simulink model "ICAC_AutoSave_20200630_1355"  (R2018b)
(part 2 of 3)

  | T_p_kPa_1_1_u8.Bias = 0;
  | T_p_kPa_1_1_u8.DataTypeOverride = 'Inherit';
  | T_p_kPa_1_1_u8.IsAlias = true;
  | 
  | T_p_kPa_256_1_u16 = Simulink.NumericType;
  | T_p_kPa_256_1_u16.Description = 'kPa (kiloPascals  (kPa))';
  | if (tmpVer > 7.11)
  | 	T_p_kPa_256_1_u16.DataScope = 'Auto';
  | end
  | T_p_kPa_256_1_u16.HeaderFile = 'Rte_Type.h';
  | T_p_kPa_256_1_u16.DataTypeMode = 'Fixed-point: slope and bias scaling';
  | T_p_kPa_256_1_u16.SignednessBool = false;
  | T_p_kPa_256_1_u16.WordLength = 16;
  | T_p_kPa_256_1_u16.FixedExponent = -8;
  | T_p_kPa_256_1_u16.SlopeAdjustmentFactor = 1;
  | T_p_kPa_256_1_u16.Bias = 0;
  | T_p_kPa_256_1_u16.DataTypeOverride = 'Inherit';
  | T_p_kPa_256_1_u16.IsAlias = true;
  | 
  | T_p_kPa_32_1_u16 = Simulink.NumericType;
  | T_p_kPa_32_1_u16.Description = 'kPa (kiloPascals  (kPa))';
  | if (tmpVer > 7.11)
  | 	T_p_kPa_32_1_u16.DataScope = 'Auto';
  | end
  | T_p_kPa_32_1_u16.HeaderFile = 'Rte_Type.h';
  | T_p_kPa_32_1_u16.DataTypeMode = 'Fixed-point: slope and bias scaling';
  | T_p_kPa_32_1_u16.SignednessBool = false;
  | T_p_kPa_32_1_u16.WordLength = 16;
  | T_p_kPa_32_1_u16.FixedExponent = -5;
  | T_p_kPa_32_1_u16.SlopeAdjustmentFactor = 1;
  | T_p_kPa_32_1_u16.Bias = 0;
  | T_p_kPa_32_1_u16.DataTypeOverride = 'Inherit';
  | T_p_kPa_32_1_u16.IsAlias = true;
  | 
  | T_p_kPa_64_1_s16 = Simulink.NumericType;
  | T_p_kPa_64_1_s16.Description = 'kPa (kiloPascals  (kPa))';
  | if (tmpVer > 7.11)
  | 	T_p_kPa_64_1_s16.DataScope = 'Auto';
  | end
  | T_p_kPa_64_1_s16.HeaderFile = 'Rte_Type.h';
  | T_p_kPa_64_1_s16.DataTypeMode = 'Fixed-point: slope and bias scaling';
  | T_p_kPa_64_1_s16.SignednessBool = true;
  | T_p_kPa_64_1_s16.WordLength = 16;
  | T_p_kPa_64_1_s16.FixedExponent = -6;
  | T_p_kPa_64_1_s16.SlopeAdjustmentFactor = 1;
  | T_p_kPa_64_1_s16.Bias = 0;
  | T_p_kPa_64_1_s16.DataTypeOverride = 'Inherit';
  | T_p_kPa_64_1_s16.IsAlias = true;
  | 
  | T_p_kPa_Float32 = Simulink.NumericType;
  | T_p_kPa_Float32.Description = 'kPa (kiloPascals  (kPa))';
  | if (tmpVer > 7.11)
  | 	T_p_kPa_Float32.DataScope = 'Auto';
  | end
  | T_p_kPa_Float32.HeaderFile = 'Rte_Type.h';
  | T_p_kPa_Float32.DataTypeMode = 'Single';
  | T_p_kPa_Float32.SignednessBool = true;
  | T_p_kPa_Float32.WordLength = 32;
  | T_p_kPa_Float32.FixedExponent = 0;
  | T_p_kPa_Float32.SlopeAdjustmentFactor = 1;
  | T_p_kPa_Float32.Bias = 0;
  | T_p_kPa_Float32.DataTypeOverride = 'Inherit';
  | T_p_kPa_Float32.IsAlias = true;
  | 
  | T_phi_deg_100_1_s16 = Simulink.NumericType;
  | T_phi_deg_100_1_s16.Description = 'deg (degrees (deg))';
  | if (tmpVer > 7.11)
  | 	T_phi_deg_100_1_s16.DataScope = 'Auto';
  | end
  | T_phi_deg_100_1_s16.HeaderFile = 'Rte_Type.h';
  | T_phi_deg_100_1_s16.DataTypeMode = ['Fixed-point: slope and bias scalin' ...
  |                                     'g'];
  | T_phi_deg_100_1_s16.SignednessBool = true;
  | T_phi_deg_100_1_s16.WordLength = 16;
  | T_phi_deg_100_1_s16.FixedExponent = -7;
  | T_phi_deg_100_1_s16.SlopeAdjustmentFactor = 1.28;
  | T_phi_deg_100_1_s16.Bias = 0;
  | T_phi_deg_100_1_s16.DataTypeOverride = 'Inherit';
  | T_phi_deg_100_1_s16.IsAlias = true;
  | 
  | T_phi_deg_1024_1_s16 = Simulink.NumericType;
  | T_phi_deg_1024_1_s16.Description = 'deg (degrees (deg))';
  | if (tmpVer > 7.11)
  | 	T_phi_deg_1024_1_s16.DataScope = 'Auto';
  | end
  | T_phi_deg_1024_1_s16.HeaderFile = 'Rte_Type.h';
  | T_phi_deg_1024_1_s16.DataTypeMode = ...
  |   'Fixed-point: slope and bias scaling';
  | T_phi_deg_1024_1_s16.SignednessBool = true;
  | T_phi_deg_1024_1_s16.WordLength = 16;
  | T_phi_deg_1024_1_s16.FixedExponent = -10;
  | T_phi_deg_1024_1_s16.SlopeAdjustmentFactor = 1;
  | T_phi_deg_1024_1_s16.Bias = 0;
  | T_phi_deg_1024_1_s16.DataTypeOverride = 'Inherit';
  | T_phi_deg_1024_1_s16.IsAlias = true;
  | 
  | T_phi_deg_128_1_s16 = Simulink.NumericType;
  | T_phi_deg_128_1_s16.Description = 'deg (degrees (deg))';
  | if (tmpVer > 7.11)
  | 	T_phi_deg_128_1_s16.DataScope = 'Auto';
  | end
  | T_phi_deg_128_1_s16.HeaderFile = 'Rte_Type.h';
  | T_phi_deg_128_1_s16.DataTypeMode = ['Fixed-point: slope and bias scalin' ...
  |                                     'g'];
  | T_phi_deg_128_1_s16.SignednessBool = true;
  | T_phi_deg_128_1_s16.WordLength = 16;
  | T_phi_deg_128_1_s16.FixedExponent = -7;
  | T_phi_deg_128_1_s16.SlopeAdjustmentFactor = 1;
  | T_phi_deg_128_1_s16.Bias = 0;
  | T_phi_deg_128_1_s16.DataTypeOverride = 'Inherit';
  | T_phi_deg_128_1_s16.IsAlias = true;
  | 
  | T_phi_deg_1_1_u8 = Simulink.NumericType;
  | T_phi_deg_1_1_u8.Description = 'deg (degrees (deg))';
  | if (tmpVer > 7.11)
  | 	T_phi_deg_1_1_u8.DataScope = 'Auto';
  | end
  | T_phi_deg_1_1_u8.HeaderFile = 'Rte_Type.h';
  | T_phi_deg_1_1_u8.DataTypeMode = 'Fixed-point: slope and bias scaling';
  | T_phi_deg_1_1_u8.SignednessBool = false;
  | T_phi_deg_1_1_u8.WordLength = 8;
  | T_phi_deg_1_1_u8.FixedExponent = 0;
  | T_phi_deg_1_1_u8.SlopeAdjustmentFactor = 1;
  | T_phi_deg_1_1_u8.Bias = 0;
  | T_phi_deg_1_1_u8.DataTypeOverride = 'Inherit';
  | T_phi_deg_1_1_u8.IsAlias = true;
  | 
  | T_phi_deg_256_1_s16 = Simulink.NumericType;
  | T_phi_deg_256_1_s16.Description = 'deg (degrees (deg))';
  | if (tmpVer > 7.11)
  | 	T_phi_deg_256_1_s16.DataScope = 'Auto';
  | end
  | T_phi_deg_256_1_s16.HeaderFile = 'Rte_Type.h';
  | T_phi_deg_256_1_s16.DataTypeMode = ['Fixed-point: slope and bias scalin' ...
  |                                     'g'];
  | T_phi_deg_256_1_s16.SignednessBool = true;
  | T_phi_deg_256_1_s16.WordLength = 16;
  | T_phi_deg_256_1_s16.FixedExponent = -8;
  | T_phi_deg_256_1_s16.SlopeAdjustmentFactor = 1;
  | T_phi_deg_256_1_s16.Bias = 0;
  | T_phi_deg_256_1_s16.DataTypeOverride = 'Inherit';
  | T_phi_deg_256_1_s16.IsAlias = true;
  | 
  | T_phi_deg_2_1_s8 = Simulink.NumericType;
  | T_phi_deg_2_1_s8.Description = 'deg (degrees (deg))';
  | if (tmpVer > 7.11)
  | 	T_phi_deg_2_1_s8.DataScope = 'Auto';
  | end
  | T_phi_deg_2_1_s8.HeaderFile = 'Rte_Type.h';
  | T_phi_deg_2_1_s8.DataTypeMode = 'Fixed-point: slope and bias scaling';
  | T_phi_deg_2_1_s8.SignednessBool = true;
  | T_phi_deg_2_1_s8.WordLength = 8;
  | T_phi_deg_2_1_s8.FixedExponent = -1;
  | T_phi_deg_2_1_s8.SlopeAdjustmentFactor = 1;
  | T_phi_deg_2_1_s8.Bias = 0;
  | T_phi_deg_2_1_s8.DataTypeOverride = 'Inherit';
  | T_phi_deg_2_1_s8.IsAlias = true;
  | 
  | T_phi_deg_32_1_s16 = Simulink.NumericType;
  | T_phi_deg_32_1_s16.Description = 'deg (degrees (deg))';
  | if (tmpVer > 7.11)
  | 	T_phi_deg_32_1_s16.DataScope = 'Auto';
  | end
  | T_phi_deg_32_1_s16.HeaderFile = 'Rte_Type.h';
  | T_phi_deg_32_1_s16.DataTypeMode = 'Fixed-point: slope and bias scaling';
  | T_phi_deg_32_1_s16.SignednessBool = true;
  | T_phi_deg_32_1_s16.WordLength = 16;
  | T_phi_deg_32_1_s16.FixedExponent = -5;
  | T_phi_deg_32_1_s16.SlopeAdjustmentFactor = 1;
  | T_phi_deg_32_1_s16.Bias = 0;
  | T_phi_deg_32_1_s16.DataTypeOverride = 'Inherit';
  | T_phi_deg_32_1_s16.IsAlias = true;
  | 
  | T_phi_deg_512_6_s32 = Simulink.NumericType;
  | T_phi_deg_512_6_s32.Description = 'deg (degrees (deg))';
  | if (tmpVer > 7.11)
  | 	T_phi_deg_512_6_s32.DataScope = 'Auto';
  | end
  | T_phi_deg_512_6_s32.HeaderFile = 'Rte_Type.h';
  | T_phi_deg_512_6_s32.DataTypeMode = ['Fixed-point: slope and bias scalin' ...
  |                                     'g'];
  | T_phi_deg_512_6_s32.SignednessBool = true;
  | T_phi_deg_512_6_s32.WordLength = 32;
  | T_phi_deg_512_6_s32.FixedExponent = -7;
  | T_phi_deg_512_6_s32.SlopeAdjustmentFactor = 1.5;
  | T_phi_deg_512_6_s32.Bias = 0;
  | T_phi_deg_512_6_s32.DataTypeOverride = 'Inherit';
  | T_phi_deg_512_6_s32.IsAlias = true;
  | 
  | T_phi_deg_Float32 = Simulink.NumericType;
  | T_phi_deg_Float32.Description = 'deg (degrees (deg))';
  | if (tmpVer > 7.11)
  | 	T_phi_deg_Float32.DataScope = 'Auto';
  | end
  | T_phi_deg_Float32.HeaderFile = 'Rte_Type.h';
  | T_phi_deg_Float32.DataTypeMode = 'Single';
  | T_phi_deg_Float32.SignednessBool = true;
  | T_phi_deg_Float32.WordLength = 32;
  | T_phi_deg_Float32.FixedExponent = 0;
  | T_phi_deg_Float32.SlopeAdjustmentFactor = 1;
  | T_phi_deg_Float32.Bias = 0;
  | T_phi_deg_Float32.DataTypeOverride = 'Inherit';
  | T_phi_deg_Float32.IsAlias = true;
  | 
  | T_phi_rad_2048_1_s16 = Simulink.NumericType;
  | T_phi_rad_2048_1_s16.Description = 'rad (radians  (rad))';
  | if (tmpVer > 7.11)
  | 	T_phi_rad_2048_1_s16.DataScope = 'Auto';
  | end
  | T_phi_rad_2048_1_s16.HeaderFile = 'Rte_Type.h';
  | T_phi_rad_2048_1_s16.DataTypeMode = ...
  |   'Fixed-point: slope and bias scaling';
  | T_phi_rad_2048_1_s16.SignednessBool = true;
  | T_phi_rad_2048_1_s16.WordLength = 16;
  | T_phi_rad_2048_1_s16.FixedExponent = -11;
  | T_phi_rad_2048_1_s16.SlopeAdjustmentFactor = 1;
  | T_phi_rad_2048_1_s16.Bias = 0;
  | T_phi_rad_2048_1_s16.DataTypeOverride = 'Inherit';
  | T_phi_rad_2048_1_s16.IsAlias = true;
  | 
  | T_phi_rad_Float32 = Simulink.NumericType;
  | T_phi_rad_Float32.Description = 'rad (radians  (rad))';
  | if (tmpVer > 7.11)
  | 	T_phi_rad_Float32.DataScope = 'Auto';
  | end
  | T_phi_rad_Float32.HeaderFile = 'Rte_Type.h';
  | T_phi_rad_Float32.DataTypeMode = 'Single';
  | T_phi_rad_Float32.SignednessBool = true;
  | T_phi_rad_Float32.WordLength = 32;
  | T_phi_rad_Float32.FixedExponent = 0;
  | T_phi_rad_Float32.SlopeAdjustmentFactor = 1;
  | T_phi_rad_Float32.Bias = 0;
  | T_phi_rad_Float32.DataTypeOverride = 'Inherit';
  | T_phi_rad_Float32.IsAlias = true;
  | 
  | T_r_NA_1024_1_s16 = Simulink.NumericType;
  | T_r_NA_1024_1_s16.Description = 'NA (none)';
  | if (tmpVer > 7.11)
  | 	T_r_NA_1024_1_s16.DataScope = 'Auto';
  | end
  | T_r_NA_1024_1_s16.HeaderFile = 'Rte_Type.h';
  | T_r_NA_1024_1_s16.DataTypeMode = 'Fixed-point: slope and bias scaling';
  | T_r_NA_1024_1_s16.SignednessBool = true;
  | T_r_NA_1024_1_s16.WordLength = 16;
  | T_r_NA_1024_1_s16.FixedExponent = -10;
  | T_r_NA_1024_1_s16.SlopeAdjustmentFactor = 1;
  | T_r_NA_1024_1_s16.Bias = 0;
  | T_r_NA_1024_1_s16.DataTypeOverride = 'Inherit';
  | T_r_NA_1024_1_s16.IsAlias = true;
  | 
  | T_r_NA_1024_1_u16 = Simulink.NumericType;
  | T_r_NA_1024_1_u16.Description = 'NA (none)';
  | if (tmpVer > 7.11)
  | 	T_r_NA_1024_1_u16.DataScope = 'Auto';
  | end
  | T_r_NA_1024_1_u16.HeaderFile = 'Rte_Type.h';
  | T_r_NA_1024_1_u16.DataTypeMode = 'Fixed-point: slope and bias scaling';
  | T_r_NA_1024_1_u16.SignednessBool = false;
  | T_r_NA_1024_1_u16.WordLength = 16;
  | T_r_NA_1024_1_u16.FixedExponent = -10;
  | T_r_NA_1024_1_u16.SlopeAdjustmentFactor = 1;
  | T_r_NA_1024_1_u16.Bias = 0;
  | T_r_NA_1024_1_u16.DataTypeOverride = 'Inherit';
  | T_r_NA_1024_1_u16.IsAlias = true;
  | 
  | T_r_NA_16384_1_s16 = Simulink.NumericType;
  | T_r_NA_16384_1_s16.Description = 'NA (none)';
  | if (tmpVer > 7.11)
  | 	T_r_NA_16384_1_s16.DataScope = 'Auto';
  | end
  | T_r_NA_16384_1_s16.HeaderFile = 'Rte_Type.h';
  | T_r_NA_16384_1_s16.DataTypeMode = 'Fixed-point: slope and bias scaling';
  | T_r_NA_16384_1_s16.SignednessBool = true;
  | T_r_NA_16384_1_s16.WordLength = 16;
  | T_r_NA_16384_1_s16.FixedExponent = -14;
  | T_r_NA_16384_1_s16.SlopeAdjustmentFactor = 1;
  | T_r_NA_16384_1_s16.Bias = 0;
  | T_r_NA_16384_1_s16.DataTypeOverride = 'Inherit';
  | T_r_NA_16384_1_s16.IsAlias = true;
  | 
  | T_r_NA_16_1_s16 = Simulink.NumericType;
  | T_r_NA_16_1_s16.Description = 'NA (none)';
  | if (tmpVer > 7.11)
  | 	T_r_NA_16_1_s16.DataScope = 'Auto';
  | end
  | T_r_NA_16_1_s16.HeaderFile = 'Rte_Type.h';
  | T_r_NA_16_1_s16.DataTypeMode = 'Fixed-point: slope and bias scaling';
  | T_r_NA_16_1_s16.SignednessBool = true;
  | T_r_NA_16_1_s16.WordLength = 16;
  | T_r_NA_16_1_s16.FixedExponent = -4;
  | T_r_NA_16_1_s16.SlopeAdjustmentFactor = 1;
  | T_r_NA_16_1_s16.Bias = 0;
  | T_r_NA_16_1_s16.DataTypeOverride = 'Inherit';
  | T_r_NA_16_1_s16.IsAlias = true;
  | 
  | T_r_NA_256_1_s8 = Simulink.NumericType;
  | T_r_NA_256_1_s8.Description = 'NA (none)';
  | if (tmpVer > 7.11)
  | 	T_r_NA_256_1_s8.DataScope = 'Auto';
  | end
  | T_r_NA_256_1_s8.HeaderFile = 'Rte_Type.h';
  | T_r_NA_256_1_s8.DataTypeMode = 'Fixed-point: slope and bias scaling';
  | T_r_NA_256_1_s8.SignednessBool = true;
  | T_r_NA_256_1_s8.WordLength = 8;
  | T_r_NA_256_1_s8.FixedExponent = -8;
  | T_r_NA_256_1_s8.SlopeAdjustmentFactor = 1;
  | T_r_NA_256_1_s8.Bias = 0;
  | T_r_NA_256_1_s8.DataTypeOverride = 'Inherit';
  | T_r_NA_256_1_s8.IsAlias = true;
  | 
  | T_r_NA_256_1_u16 = Simulink.NumericType;
  | T_r_NA_256_1_u16.Description = 'NA (none)';
  | if (tmpVer > 7.11)
  | 	T_r_NA_256_1_u16.DataScope = 'Auto';
  | end
  | T_r_NA_256_1_u16.HeaderFile = 'Rte_Type.h';
  | T_r_NA_256_1_u16.DataTypeMode = 'Fixed-point: slope and bias scaling';
  | T_r_NA_256_1_u16.SignednessBool = false;
  | T_r_NA_256_1_u16.WordLength = 16;
  | T_r_NA_256_1_u16.FixedExponent = -8;
  | T_r_NA_256_1_u16.SlopeAdjustmentFactor = 1;
  | T_r_NA_256_1_u16.Bias = 0;
  | T_r_NA_256_1_u16.DataTypeOverride = 'Inherit';
  | T_r_NA_256_1_u16.IsAlias = true;
  | 
  | T_r_NA_32768_1_u16 = Simulink.NumericType;
  | T_r_NA_32768_1_u16.Description = 'NA (none)';
  | if (tmpVer > 7.11)
  | 	T_r_NA_32768_1_u16.DataScope = 'Auto';
  | end
  | T_r_NA_32768_1_u16.HeaderFile = 'Rte_Type.h';
  | T_r_NA_32768_1_u16.DataTypeMode = 'Fixed-point: slope and bias scaling';
  | T_r_NA_32768_1_u16.SignednessBool = false;
  | T_r_NA_32768_1_u16.WordLength = 16;
  | T_r_NA_32768_1_u16.FixedExponent = -15;
  | T_r_NA_32768_1_u16.SlopeAdjustmentFactor = 1;
  | T_r_NA_32768_1_u16.Bias = 0;
  | T_r_NA_32768_1_u16.DataTypeOverride = 'Inherit';
  | T_r_NA_32768_1_u16.IsAlias = true;
  | 
  | T_r_NA_32_1_u16 = Simulink.NumericType;
  | T_r_NA_32_1_u16.Description = 'NA (none)';
  | if (tmpVer > 7.11)
  | 	T_r_NA_32_1_u16.DataScope = 'Auto';
  | end
  | T_r_NA_32_1_u16.HeaderFile = 'Rte_Type.h';
  | T_r_NA_32_1_u16.DataTypeMode = 'Fixed-point: slope and bias scaling';
  | T_r_NA_32_1_u16.SignednessBool = false;
  | T_r_NA_32_1_u16.WordLength = 16;
  | T_r_NA_32_1_u16.FixedExponent = -5;
  | T_r_NA_32_1_u16.SlopeAdjustmentFactor = 1;
  | T_r_NA_32_1_u16.Bias = 0;
  | T_r_NA_32_1_u16.DataTypeOverride = 'Inherit';
  | T_r_NA_32_1_u16.IsAlias = true;
  | 
  | T_r_NA_4096_1_s16 = Simulink.NumericType;
  | T_r_NA_4096_1_s16.Description = 'NA (none)';
  | if (tmpVer > 7.11)
  | 	T_r_NA_4096_1_s16.DataScope = 'Auto';
  | end
  | T_r_NA_4096_1_s16.HeaderFile = 'Rte_Type.h';
  | T_r_NA_4096_1_s16.DataTypeMode = 'Fixed-point: slope and bias scaling';
  | T_r_NA_4096_1_s16.SignednessBool = true;
  | T_r_NA_4096_1_s16.WordLength = 16;
  | T_r_NA_4096_1_s16.FixedExponent = -12;
  | T_r_NA_4096_1_s16.SlopeAdjustmentFactor = 1;
  | T_r_NA_4096_1_s16.Bias = 0;
  | T_r_NA_4096_1_s16.DataTypeOverride = 'Inherit';
  | T_r_NA_4096_1_s16.IsAlias = true;
  | 
  | T_r_NA_65535_2_u16 = Simulink.NumericType;
  | T_r_NA_65535_2_u16.Description = 'NA (none)';
  | if (tmpVer > 7.11)
  | 	T_r_NA_65535_2_u16.DataScope = 'Auto';
  | end
  | T_r_NA_65535_2_u16.HeaderFile = 'Rte_Type.h';
  | T_r_NA_65535_2_u16.DataTypeMode = 'Fixed-point: slope and bias scaling';
  | T_r_NA_65535_2_u16.SignednessBool = false;
  | T_r_NA_65535_2_u16.WordLength = 16;
  | T_r_NA_65535_2_u16.FixedExponent = -15;
  | T_r_NA_65535_2_u16.SlopeAdjustmentFactor = 1.0000152590218967;
  | T_r_NA_65535_2_u16.Bias = 0;
  | T_r_NA_65535_2_u16.DataTypeOverride = 'Inherit';
  | T_r_NA_65535_2_u16.IsAlias = true;
  | 
  | T_r_NA_8192_1_u16 = Simulink.NumericType;
  | T_r_NA_8192_1_u16.Description = 'NA (none)';
  | if (tmpVer > 7.11)
  | 	T_r_NA_8192_1_u16.DataScope = 'Auto';
  | end
  | T_r_NA_8192_1_u16.HeaderFile = 'Rte_Type.h';
  | T_r_NA_8192_1_u16.DataTypeMode = 'Fixed-point: slope and bias scaling';
  | T_r_NA_8192_1_u16.SignednessBool = false;
  | T_r_NA_8192_1_u16.WordLength = 16;
  | T_r_NA_8192_1_u16.FixedExponent = -13;
  | T_r_NA_8192_1_u16.SlopeAdjustmentFactor = 1;
  | T_r_NA_8192_1_u16.Bias = 0;
  | T_r_NA_8192_1_u16.DataTypeOverride = 'Inherit';
  | T_r_NA_8192_1_u16.IsAlias = true;
  | 
  | T_r_NA_Float32 = Simulink.NumericType;
  | T_r_NA_Float32.Description = 'NA (none)';
  | if (tmpVer > 7.11)
  | 	T_r_NA_Float32.DataScope = 'Auto';
  | end
  | T_r_NA_Float32.HeaderFile = 'Rte_Type.h';
  | T_r_NA_Float32.DataTypeMode = 'Single';
  | T_r_NA_Float32.SignednessBool = true;
  | T_r_NA_Float32.WordLength = 32;
  | T_r_NA_Float32.FixedExponent = 0;
  | T_r_NA_Float32.SlopeAdjustmentFactor = 1;
  | T_r_NA_Float32.Bias = 0;
  | T_r_NA_Float32.DataTypeOverride = 'Inherit';
  | T_r_NA_Float32.IsAlias = true;
  | 
  | T_rho_gpl_8192_1_s16 = Simulink.NumericType;
  | T_rho_gpl_8192_1_s16.Description = 'gpl (grams / liter  (g/l))';
  | if (tmpVer > 7.11)
  | 	T_rho_gpl_8192_1_s16.DataScope = 'Auto';
  | end
  | T_rho_gpl_8192_1_s16.HeaderFile = 'Rte_Type.h';
  | T_rho_gpl_8192_1_s16.DataTypeMode = ...
  |   'Fixed-point: slope and bias scaling';
  | T_rho_gpl_8192_1_s16.SignednessBool = true;
  | T_rho_gpl_8192_1_s16.WordLength = 16;
  | T_rho_gpl_8192_1_s16.FixedExponent = -13;
  | T_rho_gpl_8192_1_s16.SlopeAdjustmentFactor = 1;
  | T_rho_gpl_8192_1_s16.Bias = 0;
  | T_rho_gpl_8192_1_s16.DataTypeOverride = 'Inherit';
  | T_rho_gpl_8192_1_s16.IsAlias = true;
  | 
  | T_rho_gpl_Float32 = Simulink.NumericType;
  | T_rho_gpl_Float32.Description = 'gpl (grams / liter  (g/l))';
  | if (tmpVer > 7.11)
  | 	T_rho_gpl_Float32.DataScope = 'Auto';
  | end
  | T_rho_gpl_Float32.HeaderFile = 'Rte_Type.h';
  | T_rho_gpl_Float32.DataTypeMode = 'Single';
  | T_rho_gpl_Float32.SignednessBool = true;
  | T_rho_gpl_Float32.WordLength = 32;
  | T_rho_gpl_Float32.FixedExponent = 0;
  | T_rho_gpl_Float32.SlopeAdjustmentFactor = 1;
  | T_rho_gpl_Float32.Bias = 0;
  | T_rho_gpl_Float32.DataTypeOverride = 'Inherit';
  | T_rho_gpl_Float32.IsAlias = true;
  | 
  | T_rho_kgpm3_16_1_s16 = Simulink.NumericType;
  | T_rho_kgpm3_16_1_s16.Description = ['kgpm3 (kilograms / cubic meter  (k' ...
  |                                     'g/m3))'];
  | if (tmpVer > 7.11)
  | 	T_rho_kgpm3_16_1_s16.DataScope = 'Auto';
  | end
  | T_rho_kgpm3_16_1_s16.HeaderFile = 'Rte_Type.h';
  | T_rho_kgpm3_16_1_s16.DataTypeMode = ...
  |   'Fixed-point: slope and bias scaling';
  | T_rho_kgpm3_16_1_s16.SignednessBool = true;
  | T_rho_kgpm3_16_1_s16.WordLength = 16;
  | T_rho_kgpm3_16_1_s16.FixedExponent = -4;
  | T_rho_kgpm3_16_1_s16.SlopeAdjustmentFactor = 1;
  | T_rho_kgpm3_16_1_s16.Bias = 0;
  | T_rho_kgpm3_16_1_s16.DataTypeOverride = 'Inherit';
  | T_rho_kgpm3_16_1_s16.IsAlias = true;
  | 
  | T_rho_kgpm3_Float32 = Simulink.NumericType;
  | T_rho_kgpm3_Float32.Description = ['kgpm3 (kilograms / cubic meter  (kg' ...
  |                                    '/m3))'];
  | if (tmpVer > 7.11)
  | 	T_rho_kgpm3_Float32.DataScope = 'Auto';
  | end
  | T_rho_kgpm3_Float32.HeaderFile = 'Rte_Type.h';
  | T_rho_kgpm3_Float32.DataTypeMode = 'Single';
  | T_rho_kgpm3_Float32.SignednessBool = true;
  | T_rho_kgpm3_Float32.WordLength = 32;
  | T_rho_kgpm3_Float32.FixedExponent = 0;
  | T_rho_kgpm3_Float32.SlopeAdjustmentFactor = 1;
  | T_rho_kgpm3_Float32.Bias = 0;
  | T_rho_kgpm3_Float32.DataTypeOverride = 'Inherit';
  | T_rho_kgpm3_Float32.IsAlias = true;
  | 
  | T_rho_mgpl_1_1_s16 = Simulink.NumericType;
  | T_rho_mgpl_1_1_s16.Description = 'mgpl (milligrams / liter  (mg/l))';
  | if (tmpVer > 7.11)
  | 	T_rho_mgpl_1_1_s16.DataScope = 'Auto';
  | end
  | T_rho_mgpl_1_1_s16.HeaderFile = 'Rte_Type.h';
  | T_rho_mgpl_1_1_s16.DataTypeMode = 'Fixed-point: slope and bias scaling';
  | T_rho_mgpl_1_1_s16.SignednessBool = true;
  | T_rho_mgpl_1_1_s16.WordLength = 16;
  | T_rho_mgpl_1_1_s16.FixedExponent = 0;
  | T_rho_mgpl_1_1_s16.SlopeAdjustmentFactor = 1;
  | T_rho_mgpl_1_1_s16.Bias = 0;
  | T_rho_mgpl_1_1_s16.DataTypeOverride = 'Inherit';
  | T_rho_mgpl_1_1_s16.IsAlias = true;
  | 
  | T_rho_mgpl_64_1_s16 = Simulink.NumericType;
  | T_rho_mgpl_64_1_s16.Description = 'mgpl (milligrams / liter  (mg/l))';
  | if (tmpVer > 7.11)
  | 	T_rho_mgpl_64_1_s16.DataScope = 'Auto';
  | end
  | T_rho_mgpl_64_1_s16.HeaderFile = 'Rte_Type.h';
  | T_rho_mgpl_64_1_s16.DataTypeMode = ['Fixed-point: slope and bias scalin' ...
  |                                     'g'];
  | T_rho_mgpl_64_1_s16.SignednessBool = true;
  | T_rho_mgpl_64_1_s16.WordLength = 16;
  | T_rho_mgpl_64_1_s16.FixedExponent = -6;
  | T_rho_mgpl_64_1_s16.SlopeAdjustmentFactor = 1;
  | T_rho_mgpl_64_1_s16.Bias = 0;
  | T_rho_mgpl_64_1_s16.DataTypeOverride = 'Inherit';
  | T_rho_mgpl_64_1_s16.IsAlias = true;
  | 
  | T_rho_mgpl_Float32 = Simulink.NumericType;
  | T_rho_mgpl_Float32.Description = 'mgpl (milligrams / liter  (mg/l))';
  | if (tmpVer > 7.11)
  | 	T_rho_mgpl_Float32.DataScope = 'Auto';
  | end
  | T_rho_mgpl_Float32.HeaderFile = 'Rte_Type.h';
  | T_rho_mgpl_Float32.DataTypeMode = 'Single';
  | T_rho_mgpl_Float32.SignednessBool = true;
  | T_rho_mgpl_Float32.WordLength = 32;
  | T_rho_mgpl_Float32.FixedExponent = 0;
  | T_rho_mgpl_Float32.SlopeAdjustmentFactor = 1;
  | T_rho_mgpl_Float32.Bias = 0;
  | T_rho_mgpl_Float32.DataTypeOverride = 'Inherit';
  | T_rho_mgpl_Float32.IsAlias = true;
  | 
  | T_t_hour_1_1_s16 = Simulink.NumericType;
  | T_t_hour_1_1_s16.Description = 'h (hour  (h))';
  | if (tmpVer > 7.11)
  | 	T_t_hour_1_1_s16.DataScope = 'Auto';
  | end
  | T_t_hour_1_1_s16.HeaderFile = 'Rte_Type.h';
  | T_t_hour_1_1_s16.DataTypeMode = 'Fixed-point: slope and bias scaling';
  | T_t_hour_1_1_s16.SignednessBool = true;
  | T_t_hour_1_1_s16.WordLength = 16;
  | T_t_hour_1_1_s16.FixedExponent = 0;
  | T_t_hour_1_1_s16.SlopeAdjustmentFactor = 1;
  | T_t_hour_1_1_s16.Bias = 0;
  | T_t_hour_1_1_s16.DataTypeOverride = 'Inherit';
  | T_t_hour_1_1_s16.IsAlias = true;
  | 
  | T_t_hour_Float32 = Simulink.NumericType;
  | T_t_hour_Float32.Description = 'h (hour  (h))';
  | if (tmpVer > 7.11)
  | 	T_t_hour_Float32.DataScope = 'Auto';
  | end
  | T_t_hour_Float32.HeaderFile = 'Rte_Type.h';
  | T_t_hour_Float32.DataTypeMode = 'Single';
  | T_t_hour_Float32.SignednessBool = true;
  | T_t_hour_Float32.WordLength = 32;
  | T_t_hour_Float32.FixedExponent = 0;
  | T_t_hour_Float32.SlopeAdjustmentFactor = 1;
  | T_t_hour_Float32.Bias = 0;
  | T_t_hour_Float32.DataTypeOverride = 'Inherit';
  | T_t_hour_Float32.IsAlias = true;
  | 
  | T_t_m_1_1_u16 = Simulink.NumericType;
  | T_t_m_1_1_u16.Description = 'm (minutes  (m))';
  | if (tmpVer > 7.11)
  | 	T_t_m_1_1_u16.DataScope = 'Auto';
  | end
  | T_t_m_1_1_u16.HeaderFile = 'Rte_Type.h';
  | T_t_m_1_1_u16.DataTypeMode = 'Fixed-point: slope and bias scaling';
  | T_t_m_1_1_u16.SignednessBool = false;
  | T_t_m_1_1_u16.WordLength = 16;
  | T_t_m_1_1_u16.FixedExponent = 0;
  | T_t_m_1_1_u16.SlopeAdjustmentFactor = 1;
  | T_t_m_1_1_u16.Bias = 0;
  | T_t_m_1_1_u16.DataTypeOverride = 'Inherit';
  | T_t_m_1_1_u16.IsAlias = true;
  | 
  | T_t_m_Float32 = Simulink.NumericType;
  | T_t_m_Float32.Description = 'm (minutes  (m))';
  | if (tmpVer > 7.11)
  | 	T_t_m_Float32.DataScope = 'Auto';
  | end
  | T_t_m_Float32.HeaderFile = 'Rte_Type.h';
  | T_t_m_Float32.DataTypeMode = 'Single';
  | T_t_m_Float32.SignednessBool = true;
  | T_t_m_Float32.WordLength = 32;
  | T_t_m_Float32.FixedExponent = 0;
  | T_t_m_Float32.SlopeAdjustmentFactor = 1;
  | T_t_m_Float32.Bias = 0;
  | T_t_m_Float32.DataTypeOverride = 'Inherit';
  | T_t_m_Float32.IsAlias = true;
  | 
  | T_t_ms_1_1_s16 = Simulink.NumericType;
  | T_t_ms_1_1_s16.Description = 'ms (milliseconds  (ms))';
  | if (tmpVer > 7.11)
  | 	T_t_ms_1_1_s16.DataScope = 'Auto';
  | end
  | T_t_ms_1_1_s16.HeaderFile = 'Rte_Type.h';
  | T_t_ms_1_1_s16.DataTypeMode = 'Fixed-point: slope and bias scaling';
  | T_t_ms_1_1_s16.SignednessBool = true;
  | T_t_ms_1_1_s16.WordLength = 16;
  | T_t_ms_1_1_s16.FixedExponent = 0;
  | T_t_ms_1_1_s16.SlopeAdjustmentFactor = 1;
  | T_t_ms_1_1_s16.Bias = 0;
  | T_t_ms_1_1_s16.DataTypeOverride = 'Inherit';
  | T_t_ms_1_1_s16.IsAlias = true;
  | 
  | T_t_ms_1_1_u16 = Simulink.NumericType;
  | T_t_ms_1_1_u16.Description = 'ms (milliseconds  (ms))';
  | if (tmpVer > 7.11)
  | 	T_t_ms_1_1_u16.DataScope = 'Auto';
  | end
  | T_t_ms_1_1_u16.HeaderFile = 'Rte_Type.h';
  | T_t_ms_1_1_u16.DataTypeMode = 'Fixed-point: slope and bias scaling';
  | T_t_ms_1_1_u16.SignednessBool = false;
  | T_t_ms_1_1_u16.WordLength = 16;
  | T_t_ms_1_1_u16.FixedExponent = 0;
  | T_t_ms_1_1_u16.SlopeAdjustmentFactor = 1;
  | T_t_ms_1_1_u16.Bias = 0;
  | T_t_ms_1_1_u16.DataTypeOverride = 'Inherit';
  | T_t_ms_1_1_u16.IsAlias = true;
  | 
  | T_t_ms_1_1_u32 = Simulink.NumericType;
  | T_t_ms_1_1_u32.Description = 'ms (milliseconds  (ms))';
  | if (tmpVer > 7.11)
  | 	T_t_ms_1_1_u32.DataScope = 'Auto';
  | end
  | T_t_ms_1_1_u32.HeaderFile = 'Rte_Type.h';
  | T_t_ms_1_1_u32.DataTypeMode = 'Fixed-point: slope and bias scaling';
  | T_t_ms_1_1_u32.SignednessBool = false;
  | T_t_ms_1_1_u32.WordLength = 32;
  | T_t_ms_1_1_u32.FixedExponent = 0;
  | T_t_ms_1_1_u32.SlopeAdjustmentFactor = 1;
  | T_t_ms_1_1_u32.Bias = 0;
  | T_t_ms_1_1_u32.DataTypeOverride = 'Inherit';
  | T_t_ms_1_1_u32.IsAlias = true;
  | 
  | T_t_ms_4096_1_s16 = Simulink.NumericType;
  | T_t_ms_4096_1_s16.Description = 'ms (milliseconds  (ms))';
  | if (tmpVer > 7.11)
  | 	T_t_ms_4096_1_s16.DataScope = 'Auto';
  | end
  | T_t_ms_4096_1_s16.HeaderFile = 'Rte_Type.h';
  | T_t_ms_4096_1_s16.DataTypeMode = 'Fixed-point: slope and bias scaling';
  | T_t_ms_4096_1_s16.SignednessBool = true;
  | T_t_ms_4096_1_s16.WordLength = 16;
  | T_t_ms_4096_1_s16.FixedExponent = -12;
  | T_t_ms_4096_1_s16.SlopeAdjustmentFactor = 1;
  | T_t_ms_4096_1_s16.Bias = 0;
  | T_t_ms_4096_1_s16.DataTypeOverride = 'Inherit';
  | T_t_ms_4096_1_s16.IsAlias = true;
  | 
  | T_t_ms_64_1_s16 = Simulink.NumericType;
  | T_t_ms_64_1_s16.Description = 'ms (milliseconds  (ms))';
  | if (tmpVer > 7.11)
  | 	T_t_ms_64_1_s16.DataScope = 'Auto';
  | end
  | T_t_ms_64_1_s16.HeaderFile = 'Rte_Type.h';
  | T_t_ms_64_1_s16.DataTypeMode = 'Fixed-point: slope and bias scaling';
  | T_t_ms_64_1_s16.SignednessBool = true;
  | T_t_ms_64_1_s16.WordLength = 16;
  | T_t_ms_64_1_s16.FixedExponent = -6;
  | T_t_ms_64_1_s16.SlopeAdjustmentFactor = 1;
  | T_t_ms_64_1_s16.Bias = 0;
  | T_t_ms_64_1_s16.DataTypeOverride = 'Inherit';
  | T_t_ms_64_1_s16.IsAlias = true;
  | 
  | T_t_ms_Float32 = Simulink.NumericType;
  | T_t_ms_Float32.Description = 'ms (milliseconds  (ms))';
  | if (tmpVer > 7.11)
  | 	T_t_ms_Float32.DataScope = 'Auto';
  | end
  | T_t_ms_Float32.HeaderFile = 'Rte_Type.h';
  | T_t_ms_Float32.DataTypeMode = 'Single';
  | T_t_ms_Float32.SignednessBool = true;
  | T_t_ms_Float32.WordLength = 32;
  | T_t_ms_Float32.FixedExponent = 0;
  | T_t_ms_Float32.SlopeAdjustmentFactor = 1;
  | T_t_ms_Float32.Bias = 0;
  | T_t_ms_Float32.DataTypeOverride = 'Inherit';
  | T_t_ms_Float32.IsAlias = true;
  | 
  | T_t_s_1000_1_s16 = Simulink.NumericType;
  | T_t_s_1000_1_s16.Description = 's (seconds  (s))';
  | if (tmpVer > 7.11)
  | 	T_t_s_1000_1_s16.DataScope = 'Auto';
  | end
  | T_t_s_1000_1_s16.HeaderFile = 'Rte_Type.h';
  | T_t_s_1000_1_s16.DataTypeMode = 'Fixed-point: slope and bias scaling';
  | T_t_s_1000_1_s16.SignednessBool = true;
  | T_t_s_1000_1_s16.WordLength = 16;
  | T_t_s_1000_1_s16.FixedExponent = -10;
  | T_t_s_1000_1_s16.SlopeAdjustmentFactor = 1.024;
  | T_t_s_1000_1_s16.Bias = 0;
  | T_t_s_1000_1_s16.DataTypeOverride = 'Inherit';
  | T_t_s_1000_1_s16.IsAlias = true;
  | 
  | T_t_s_100_1_s16 = Simulink.NumericType;
  | T_t_s_100_1_s16.Description = 's (seconds  (s))';
  | if (tmpVer > 7.11)
  | 	T_t_s_100_1_s16.DataScope = 'Auto';
  | end
  | T_t_s_100_1_s16.HeaderFile = 'Rte_Type.h';
  | T_t_s_100_1_s16.DataTypeMode = 'Fixed-point: slope and bias scaling';
  | T_t_s_100_1_s16.SignednessBool = true;
  | T_t_s_100_1_s16.WordLength = 16;
  | T_t_s_100_1_s16.FixedExponent = -7;
  | T_t_s_100_1_s16.SlopeAdjustmentFactor = 1.28;
  | T_t_s_100_1_s16.Bias = 0;
  | T_t_s_100_1_s16.DataTypeOverride = 'Inherit';
  | T_t_s_100_1_s16.IsAlias = true;
  | 
  | T_t_s_10_1_s16 = Simulink.NumericType;
  | T_t_s_10_1_s16.Description = 's (seconds  (s))';
  | if (tmpVer > 7.11)
  | 	T_t_s_10_1_s16.DataScope = 'Auto';
  | end
  | T_t_s_10_1_s16.HeaderFile = 'Rte_Type.h';
  | T_t_s_10_1_s16.DataTypeMode = 'Fixed-point: slope and bias scaling';
  | T_t_s_10_1_s16.SignednessBool = true;
  | T_t_s_10_1_s16.WordLength = 16;
  | T_t_s_10_1_s16.FixedExponent = -4;
  | T_t_s_10_1_s16.SlopeAdjustmentFactor = 1.6;
  | T_t_s_10_1_s16.Bias = 0;
  | T_t_s_10_1_s16.DataTypeOverride = 'Inherit';
  | T_t_s_10_1_s16.IsAlias = true;
  | 
  | T_t_s_10_1_u16 = Simulink.NumericType;
  | T_t_s_10_1_u16.Description = 's (seconds  (s))';
  | if (tmpVer > 7.11)
  | 	T_t_s_10_1_u16.DataScope = 'Auto';
  | end
  | T_t_s_10_1_u16.HeaderFile = 'Rte_Type.h';
  | T_t_s_10_1_u16.DataTypeMode = 'Fixed-point: slope and bias scaling';
  | T_t_s_10_1_u16.SignednessBool = false;
  | T_t_s_10_1_u16.WordLength = 16;
  | T_t_s_10_1_u16.FixedExponent = -4;
  | T_t_s_10_1_u16.SlopeAdjustmentFactor = 1.6;
  | T_t_s_10_1_u16.Bias = 0;
  | T_t_s_10_1_u16.DataTypeOverride = 'Inherit';
  | T_t_s_10_1_u16.IsAlias = true;
  | 
  | T_t_s_1_1_s16 = Simulink.NumericType;
  | T_t_s_1_1_s16.Description = 's (seconds  (s))';
  | if (tmpVer > 7.11)
  | 	T_t_s_1_1_s16.DataScope = 'Auto';
  | end
  | T_t_s_1_1_s16.HeaderFile = 'Rte_Type.h';
  | T_t_s_1_1_s16.DataTypeMode = 'Fixed-point: slope and bias scaling';
  | T_t_s_1_1_s16.SignednessBool = true;
  | T_t_s_1_1_s16.WordLength = 16;
  | T_t_s_1_1_s16.FixedExponent = 0;
  | T_t_s_1_1_s16.SlopeAdjustmentFactor = 1;
  | T_t_s_1_1_s16.Bias = 0;
  | T_t_s_1_1_s16.DataTypeOverride = 'Inherit';
  | T_t_s_1_1_s16.IsAlias = true;
  | 
  | T_t_s_1_1_u16 = Simulink.NumericType;
  | T_t_s_1_1_u16.Description = 's (seconds  (s))';
  | if (tmpVer > 7.11)
  | 	T_t_s_1_1_u16.DataScope = 'Auto';
  | end
  | T_t_s_1_1_u16.HeaderFile = 'Rte_Type.h';
  | T_t_s_1_1_u16.DataTypeMode = 'Fixed-point: slope and bias scaling';
  | T_t_s_1_1_u16.SignednessBool = false;
  | T_t_s_1_1_u16.WordLength = 16;
  | T_t_s_1_1_u16.FixedExponent = 0;
  | T_t_s_1_1_u16.SlopeAdjustmentFactor = 1;
  | T_t_s_1_1_u16.Bias = 0;
  | T_t_s_1_1_u16.DataTypeOverride = 'Inherit';
  | T_t_s_1_1_u16.IsAlias = true;
  | 
  | T_t_s_1_1_u32 = Simulink.NumericType;
  | T_t_s_1_1_u32.Description = 's (seconds  (s))';
  | if (tmpVer > 7.11)
  | 	T_t_s_1_1_u32.DataScope = 'Auto';
  | end
  | T_t_s_1_1_u32.HeaderFile = 'Rte_Type.h';
  | T_t_s_1_1_u32.DataTypeMode = 'Fixed-point: slope and bias scaling';
  | T_t_s_1_1_u32.SignednessBool = false;
  | T_t_s_1_1_u32.WordLength = 32;
  | T_t_s_1_1_u32.FixedExponent = 0;
  | T_t_s_1_1_u32.SlopeAdjustmentFactor = 1;
  | T_t_s_1_1_u32.Bias = 0;
  | T_t_s_1_1_u32.DataTypeOverride = 'Inherit';
  | T_t_s_1_1_u32.IsAlias = true;
  | 
  | T_t_s_Float32 = Simulink.NumericType;
  | T_t_s_Float32.Description = 's (seconds  (s))';
  | if (tmpVer > 7.11)
  | 	T_t_s_Float32.DataScope = 'Auto';
  | end
  | T_t_s_Float32.HeaderFile = 'Rte_Type.h';
  | T_t_s_Float32.DataTypeMode = 'Single';
  | T_t_s_Float32.SignednessBool = true;
  | T_t_s_Float32.WordLength = 32;
  | T_t_s_Float32.FixedExponent = 0;
  | T_t_s_Float32.SlopeAdjustmentFactor = 1;
  | T_t_s_Float32.Bias = 0;
  | T_t_s_Float32.DataTypeOverride = 'Inherit';
  | T_t_s_Float32.IsAlias = true;
  | 
  | T_t_us_10_1_u32 = Simulink.NumericType;
  | T_t_us_10_1_u32.Description = 'us (microseconds  (us))';
  | if (tmpVer > 7.11)
  | 	T_t_us_10_1_u32.DataScope = 'Auto';
  | end
  | T_t_us_10_1_u32.HeaderFile = 'Rte_Type.h';
  | T_t_us_10_1_u32.DataTypeMode = 'Fixed-point: slope and bias scaling';
  | T_t_us_10_1_u32.SignednessBool = false;
  | T_t_us_10_1_u32.WordLength = 32;
  | T_t_us_10_1_u32.FixedExponent = -4;
  | T_t_us_10_1_u32.SlopeAdjustmentFactor = 1.6;
  | T_t_us_10_1_u32.Bias = 0;
  | T_t_us_10_1_u32.DataTypeOverride = 'Inherit';
  | T_t_us_10_1_u32.IsAlias = true;
  | 
  | T_t_us_1_1_s16 = Simulink.NumericType;
  | T_t_us_1_1_s16.Description = 'us (microseconds  (us))';
  | if (tmpVer > 7.11)
  | 	T_t_us_1_1_s16.DataScope = 'Auto';
  | end
  | T_t_us_1_1_s16.HeaderFile = 'Rte_Type.h';
  | T_t_us_1_1_s16.DataTypeMode = 'Fixed-point: slope and bias scaling';
  | T_t_us_1_1_s16.SignednessBool = true;
  | T_t_us_1_1_s16.WordLength = 16;
  | T_t_us_1_1_s16.FixedExponent = 0;
  | T_t_us_1_1_s16.SlopeAdjustmentFactor = 1;
  | T_t_us_1_1_s16.Bias = 0;
  | T_t_us_1_1_s16.DataTypeOverride = 'Inherit';
  | T_t_us_1_1_s16.IsAlias = true;
  | 
  | T_t_us_1_1_u32 = Simulink.NumericType;
  | T_t_us_1_1_u32.Description = 'us (microseconds  (us))';
  | if (tmpVer > 7.11)
  | 	T_t_us_1_1_u32.DataScope = 'Auto';
  | end
  | T_t_us_1_1_u32.HeaderFile = 'Rte_Type.h';
  | T_t_us_1_1_u32.DataTypeMode = 'Fixed-point: slope and bias scaling';
  | T_t_us_1_1_u32.SignednessBool = false;
  | T_t_us_1_1_u32.WordLength = 32;
  | T_t_us_1_1_u32.FixedExponent = 0;
  | T_t_us_1_1_u32.SlopeAdjustmentFactor = 1;
  | T_t_us_1_1_u32.Bias = 0;
  | T_t_us_1_1_u32.DataTypeOverride = 'Inherit';
  | T_t_us_1_1_u32.IsAlias = true;
  | 
  | T_t_us_1_4_u16 = Simulink.NumericType;
  | T_t_us_1_4_u16.Description = 'us (microseconds  (us))';
  | if (tmpVer > 7.11)
  | 	T_t_us_1_4_u16.DataScope = 'Auto';
  | end
  | T_t_us_1_4_u16.HeaderFile = 'Rte_Type.h';
  | T_t_us_1_4_u16.DataTypeMode = 'Fixed-point: slope and bias scaling';
  | T_t_us_1_4_u16.SignednessBool = false;
  | T_t_us_1_4_u16.WordLength = 16;
  | T_t_us_1_4_u16.FixedExponent = 2;
  | T_t_us_1_4_u16.SlopeAdjustmentFactor = 1;
  | T_t_us_1_4_u16.Bias = 0;
  | T_t_us_1_4_u16.DataTypeOverride = 'Inherit';
  | T_t_us_1_4_u16.IsAlias = true;
  | 
  | T_t_us_Float32 = Simulink.NumericType;
  | T_t_us_Float32.Description = 'us (microseconds  (us))';
  | if (tmpVer > 7.11)
  | 	T_t_us_Float32.DataScope = 'Auto';
  | end
  | T_t_us_Float32.HeaderFile = 'Rte_Type.h';
  | T_t_us_Float32.DataTypeMode = 'Single';
  | T_t_us_Float32.SignednessBool = true;
  | T_t_us_Float32.WordLength = 32;
  | T_t_us_Float32.FixedExponent = 0;
  | T_t_us_Float32.SlopeAdjustmentFactor = 1;
  | T_t_us_Float32.Bias = 0;
  | T_t_us_Float32.DataTypeOverride = 'Inherit';
  | T_t_us_Float32.IsAlias = true;
  | 
  | T_v_kph_1_1_u8 = Simulink.NumericType;
  | T_v_kph_1_1_u8.Description = 'kph (kilometers / hour  (kph))';
  | if (tmpVer > 7.11)
  | 	T_v_kph_1_1_u8.DataScope = 'Auto';
  | end
  | T_v_kph_1_1_u8.HeaderFile = 'Rte_Type.h';
  | T_v_kph_1_1_u8.DataTypeMode = 'Fixed-point: slope and bias scaling';
  | T_v_kph_1_1_u8.SignednessBool = false;
  | T_v_kph_1_1_u8.WordLength = 8;
  | T_v_kph_1_1_u8.FixedExponent = 0;
  | T_v_kph_1_1_u8.SlopeAdjustmentFactor = 1;
  | T_v_kph_1_1_u8.Bias = 0;
  | T_v_kph_1_1_u8.DataTypeOverride = 'Inherit';
  | T_v_kph_1_1_u8.IsAlias = true;
  | 
  | T_v_kph_64_1_s16 = Simulink.NumericType;
  | T_v_kph_64_1_s16.Description = 'kph (kilometers / hour  (kph))';
  | if (tmpVer > 7.11)
  | 	T_v_kph_64_1_s16.DataScope = 'Auto';
  | end
  | T_v_kph_64_1_s16.HeaderFile = 'Rte_Type.h';
  | T_v_kph_64_1_s16.DataTypeMode = 'Fixed-point: slope and bias scaling';
  | T_v_kph_64_1_s16.SignednessBool = true;
  | T_v_kph_64_1_s16.WordLength = 16;
  | T_v_kph_64_1_s16.FixedExponent = -6;
  | T_v_kph_64_1_s16.SlopeAdjustmentFactor = 1;
  | T_v_kph_64_1_s16.Bias = 0;
  | T_v_kph_64_1_s16.DataTypeOverride = 'Inherit';
  | T_v_kph_64_1_s16.IsAlias = true;
  | 
  | T_v_kph_64_1_u16 = Simulink.NumericType;
  | T_v_kph_64_1_u16.Description = 'kph (kilometers / hour  (kph))';
  | if (tmpVer > 7.11)
  | 	T_v_kph_64_1_u16.DataScope = 'Auto';
  | end
  | T_v_kph_64_1_u16.HeaderFile = 'Rte_Type.h';
  | T_v_kph_64_1_u16.DataTypeMode = 'Fixed-point: slope and bias scaling';
  | T_v_kph_64_1_u16.SignednessBool = false;
  | T_v_kph_64_1_u16.WordLength = 16;
  | T_v_kph_64_1_u16.FixedExponent = -6;
  | T_v_kph_64_1_u16.SlopeAdjustmentFactor = 1;
  | T_v_kph_64_1_u16.Bias = 0;
  | T_v_kph_64_1_u16.DataTypeOverride = 'Inherit';
  | T_v_kph_64_1_u16.IsAlias = true;
  | 
  | T_v_kph_Float32 = Simulink.NumericType;
  | T_v_kph_Float32.Description = 'kph (kilometers / hour  (kph))';
  | if (tmpVer > 7.11)
  | 	T_v_kph_Float32.DataScope = 'Auto';
  | end
  | T_v_kph_Float32.HeaderFile = 'Rte_Type.h';
  | T_v_kph_Float32.DataTypeMode = 'Single';
  | T_v_kph_Float32.SignednessBool = true;
  | T_v_kph_Float32.WordLength = 32;
  | T_v_kph_Float32.FixedExponent = 0;
  | T_v_kph_Float32.SlopeAdjustmentFactor = 1;
  | T_v_kph_Float32.Bias = 0;
  | T_v_kph_Float32.DataTypeOverride = 'Inherit';
  | T_v_kph_Float32.IsAlias = true;
  | 
  | T_v_mps_256_1_s16 = Simulink.NumericType;
  | T_v_mps_256_1_s16.Description = 'mps (meters / second  (m/s))';
  | if (tmpVer > 7.11)
  | 	T_v_mps_256_1_s16.DataScope = 'Auto';
  | end
  | T_v_mps_256_1_s16.HeaderFile = 'Rte_Type.h';
  | T_v_mps_256_1_s16.DataTypeMode = 'Fixed-point: slope and bias scaling';
  | T_v_mps_256_1_s16.SignednessBool = true;
  | T_v_mps_256_1_s16.WordLength = 16;
  | T_v_mps_256_1_s16.FixedExponent = -8;
  | T_v_mps_256_1_s16.SlopeAdjustmentFactor = 1;
  | T_v_mps_256_1_s16.Bias = 0;
  | T_v_mps_256_1_s16.DataTypeOverride = 'Inherit';
  | T_v_mps_256_1_s16.IsAlias = true;
  | 
  | T_v_mps_Float32 = Simulink.NumericType;
  | T_v_mps_Float32.Description = 'mps (meters / second  (m/s))';
  | if (tmpVer > 7.11)
  | 	T_v_mps_Float32.DataScope = 'Auto';
  | end
  | T_v_mps_Float32.HeaderFile = 'Rte_Type.h';
  | T_v_mps_Float32.DataTypeMode = 'Single';
  | T_v_mps_Float32.SignednessBool = true;
  | T_v_mps_Float32.WordLength = 32;
  | T_v_mps_Float32.FixedExponent = 0;
  | T_v_mps_Float32.SlopeAdjustmentFactor = 1;
  | T_v_mps_Float32.Bias = 0;
  | T_v_mps_Float32.DataTypeOverride = 'Inherit';
  | T_v_mps_Float32.IsAlias = true;
  | 
  | T_w_radps_32_1_s16 = Simulink.NumericType;
  | T_w_radps_32_1_s16.Description = 'radps (radians / second  (rad/s))';
  | if (tmpVer > 7.11)
  | 	T_w_radps_32_1_s16.DataScope = 'Auto';
  | end
  | T_w_radps_32_1_s16.HeaderFile = 'Rte_Type.h';
  | T_w_radps_32_1_s16.DataTypeMode = 'Fixed-point: slope and bias scaling';
  | T_w_radps_32_1_s16.SignednessBool = true;
  | T_w_radps_32_1_s16.WordLength = 16;
  | T_w_radps_32_1_s16.FixedExponent = -5;
  | T_w_radps_32_1_s16.SlopeAdjustmentFactor = 1;
  | T_w_radps_32_1_s16.Bias = 0;
  | T_w_radps_32_1_s16.DataTypeOverride = 'Inherit';
  | T_w_radps_32_1_s16.IsAlias = true;
  | 
  | T_w_radps_Float32 = Simulink.NumericType;
  | T_w_radps_Float32.Description = 'radps (radians / second  (rad/s))';
  | if (tmpVer > 7.11)
  | 	T_w_radps_Float32.DataScope = 'Auto';
  | end
  | T_w_radps_Float32.HeaderFile = 'Rte_Type.h';
  | T_w_radps_Float32.DataTypeMode = 'Single';
  | T_w_radps_Float32.SignednessBool = true;
  | T_w_radps_Float32.WordLength = 32;
  | T_w_radps_Float32.FixedExponent = 0;
  | T_w_radps_Float32.SlopeAdjustmentFactor = 1;
  | T_w_radps_Float32.Bias = 0;
  | T_w_radps_Float32.DataTypeOverride = 'Inherit';
  | T_w_radps_Float32.IsAlias = true;
  | 
  | T_y_BitField8 = Simulink.NumericType;
  | T_y_BitField8.Description = 'BitField';
  | if (tmpVer > 7.11)
  | 	T_y_BitField8.DataScope = 'Auto';
  | end
  | T_y_BitField8.HeaderFile = 'Rte_Type.h';
  | T_y_BitField8.DataTypeMode = 'Fixed-point: slope and bias scaling';
  | T_y_BitField8.SignednessBool = false;
  | T_y_BitField8.WordLength = 8;
  | T_y_BitField8.FixedExponent = 0;
  | T_y_BitField8.SlopeAdjustmentFactor = 1;
  | T_y_BitField8.Bias = 0;
  | T_y_BitField8.DataTypeOverride = 'Inherit';
  | T_y_BitField8.IsAlias = true;
  | 
  | T_y_BitFieldDiagProgress = Simulink.NumericType;
  | T_y_BitFieldDiagProgress.Description = 'BitField';
  | if (tmpVer > 7.11)
  | 	T_y_BitFieldDiagProgress.DataScope = 'Auto';
  | end
  | T_y_BitFieldDiagProgress.HeaderFile = 'Rte_Type.h';
  | T_y_BitFieldDiagProgress.DataTypeMode = ...
  |   'Fixed-point: slope and bias scaling';
  | T_y_BitFieldDiagProgress.SignednessBool = false;
  | T_y_BitFieldDiagProgress.WordLength = 8;
  | T_y_BitFieldDiagProgress.FixedExponent = 0;
  | T_y_BitFieldDiagProgress.SlopeAdjustmentFactor = 1;
  | T_y_BitFieldDiagProgress.Bias = 0;
  | T_y_BitFieldDiagProgress.DataTypeOverride = 'Inherit';
  | T_y_BitFieldDiagProgress.IsAlias = true;
  | 
  | T_y_BitFieldDiagStatus = Simulink.NumericType;
  | T_y_BitFieldDiagStatus.Description = 'BitField';
  | if (tmpVer > 7.11)
  | 	T_y_BitFieldDiagStatus.DataScope = 'Auto';
  | end
  | T_y_BitFieldDiagStatus.HeaderFile = 'Rte_Type.h';
  | T_y_BitFieldDiagStatus.DataTypeMode = ...
  |   'Fixed-point: slope and bias scaling';
  | T_y_BitFieldDiagStatus.SignednessBool = false;
  | T_y_BitFieldDiagStatus.WordLength = 8;
  | T_y_BitFieldDiagStatus.FixedExponent = 0;
  | T_y_BitFieldDiagStatus.SlopeAdjustmentFactor = 1;
  | T_y_BitFieldDiagStatus.Bias = 0;
  | T_y_BitFieldDiagStatus.DataTypeOverride = 'Inherit';
  | T_y_BitFieldDiagStatus.IsAlias = true;
  | 
  | T_y_NA_1_1_u8 = Simulink.NumericType;
  | T_y_NA_1_1_u8.Description = 'TYPE TO BE REMOVED';
  | if (tmpVer > 7.11)
  | 	T_y_NA_1_1_u8.DataScope = 'Auto';
  | end
  | T_y_NA_1_1_u8.HeaderFile = 'Rte_Type.h';
  | T_y_NA_1_1_u8.DataTypeMode = 'Fixed-point: slope and bias scaling';
  | T_y_NA_1_1_u8.SignednessBool = false;
  | T_y_NA_1_1_u8.WordLength = 8;
  | T_y_NA_1_1_u8.FixedExponent = 0;
  | T_y_NA_1_1_u8.SlopeAdjustmentFactor = 1;
  | T_y_NA_1_1_u8.Bias = 0;
  | T_y_NA_1_1_u8.DataTypeOverride = 'Inherit';
  | T_y_NA_1_1_u8.IsAlias = true;
  | 
  | UInt16 = Simulink.AliasType;
  | UInt16.Description = 'Num';
  | if (tmpVer > 7.11)
  | 	UInt16.DataScope = 'Auto';
  | end
  | UInt16.HeaderFile = 'Rte_Type.h';
  | UInt16.BaseType = 'uint16';
  | 
  | UInt32 = Simulink.AliasType;
  | UInt32.Description = 'Num';
  | if (tmpVer > 7.11)
  | 	UInt32.DataScope = 'Auto';
  | end
  | UInt32.HeaderFile = 'Rte_Type.h';
  | UInt32.BaseType = 'uint32';
  | 
  | UInt8 = Simulink.AliasType;
  | UInt8.Description = 'Num';
  | if (tmpVer > 7.11)
  | 	UInt8.DataScope = 'Auto';
  | end
  | UInt8.HeaderFile = 'Rte_Type.h';
  | UInt8.BaseType = 'uint8';
  | 
  | s16 = Simulink.AliasType;
  | s16.Description = 'TYPE TO BE REMOVED';
  | if (tmpVer > 7.11)
  | 	s16.DataScope = 'Auto';
  | end
  | s16.HeaderFile = 'Rte_Type.h';
  | s16.BaseType = 'int16';
  | 
  | s32 = Simulink.AliasType;
  | s32.Description = 'TYPE TO BE REMOVED';
  | if (tmpVer > 7.11)
  | 	s32.DataScope = 'Auto';
  | end
  | s32.HeaderFile = 'Rte_Type.h';
  | s32.BaseType = 'int32';
  | 
  | s8 = Simulink.AliasType;
  | s8.Description = 'TYPE TO BE REMOVED';
  | if (tmpVer > 7.11)
  | 	s8.DataScope = 'Auto';
  | end
  | s8.HeaderFile = 'Rte_Type.h';
  | s8.BaseType = 'int8';
  | 
  | u16 = Simulink.AliasType;
  | u16.Description = 'TYPE TO BE REMOVED';
  | if (tmpVer > 7.11)
  | 	u16.DataScope = 'Auto';
  | end
  | u16.HeaderFile = 'Rte_Type.h';
  | u16.BaseType = 'uint16';
  | 
  | u32 = Simulink.AliasType;
  | u32.Description = 'TYPE TO BE REMOVED';
  | if (tmpVer > 7.11)
  | 	u32.DataScope = 'Auto';
  | end
  | u32.HeaderFile = 'Rte_Type.h';
  | u32.BaseType = 'uint32';
  | 
  | u8 = Simulink.AliasType;
  | u8.Description = 'TYPE TO BE REMOVED';
  | if (tmpVer > 7.11)
  | 	u8.DataScope = 'Auto';
  | end
  | u8.HeaderFile = 'Rte_Type.h';
  | u8.BaseType = 'uint8';
  | 
  | clear tmpVer
StopFcn:
  | clear  T_A_m2_1024_1_u32 T_A_m2_65536_1_u16 T_A_m2_Float32 T_A_mm2_10_1_u16 T_A_mm2_4_1_s16 T_A_mm2_Float32 T_Cnt_Num_10_1_u32 T_Cnt_Num_1_1_s16 T_Cnt_Num_1_1_s32 T_Cnt_Num_1_1_s8 T_Cnt_Num_1_1_u16 T_Cnt_Num_1_1_u32 T_Cnt_Num_1_1_u8 T_E_J_1_1_s32 T_E_J_Float32 T_E_kJ_128_1_s32 T_E_kJ_Float32 T_E_kwh_10_1_u16 T_E_kwh_Float32 T_Epl_kwhpkm_100_1_u16 T_Epl_kwhpkm_Float32 T_F_N_1_1_s16 T_F_N_Float32 T_I_A_1000_1_u16 T_I_A_1048576_1_s32 T_I_A_2048_1_s16 T_I_A_32_1_s16 T_I_A_Float32 T_I_mA_1_1_s16 T_I_mA_32768_128_s16 T_I_mA_Float32 T_J_kgpm2_128_1_u16 T_J_kgpm2_Float32 T_K_NA_1000_1_s16 T_K_NA_100_1_s16 T_K_NA_100_1_u16 T_K_NA_1024_1_s16 T_K_NA_1024_1_u16 T_K_NA_128_1_s16 T_K_NA_128_1_u16 T_K_NA_128_1_u8 T_K_NA_16777216_1_u32 T_K_NA_16_1_s16 T_K_NA_16_1_u16 T_K_NA_16_1_u8 T_K_NA_1_16_u16 T_K_NA_1_1_s16 T_K_NA_1_1_u16 T_K_NA_1_1_u8 T_K_NA_32768_1_s16 T_K_NA_32768_1_u16 T_K_NA_32_1_s8 T_K_NA_4096_1_u16 T_K_NA_4194304_1_s32 T_K_NA_4194304_1_u16 T_K_NA_65536_1_s32 T_K_NA_65536_1_u16 T_K_NA_8192_1_s16 T_K_NA_8_1_s16 T_K_NA_Float32 T_M_Nm_16_1_s16 T_M_Nm_1_1_s16 T_M_Nm_32768_1_s16 T_M_Nm_32_1_s16 T_M_Nm_4_1_s16 T_M_Nm_512_1_s16 T_M_Nm_Float32 T_P_W_1_4_s16 T_P_W_1_8_s16 T_P_W_Float32 T_P_kW_128_1_s16 T_P_kW_1_8_s16 T_P_kW_8_1_s32 T_P_kW_Float32 T_Pct_pct_1024_1_s32 T_Pct_pct_1024_1_u32 T_Pct_pct_10_1_s16 T_Pct_pct_10_1_u32 T_Pct_pct_128_100_s8 T_Pct_pct_1_1_s16 T_Pct_pct_1_4_u8 T_Pct_pct_255_100_u16 T_Pct_pct_255_100_u8 T_Pct_pct_256_1_s16 T_Pct_pct_256_1_u16 T_Pct_pct_65535_100_u16 T_Pct_pct_Float32 T_R_ohm_1024_1_s16 T_R_ohm_32_1_s16 T_R_ohm_Float32 T_TK_K_16_1_s16 T_TK_K_Float32 T_T_degC_10_400_1_u16 T_T_degC_16_1_s16 T_T_degC_1_40_1_u8 T_T_degC_2_80_1_u8 T_T_degC_Float32 T_U_V_1000_1_u16 T_U_V_10_1_u8 T_U_V_200_1_u8 T_U_V_32_1_s16 T_U_V_4096_1_s16 T_U_V_512_1_s16 T_U_V_65535_8_u16 T_U_V_8192_1_u16 T_U_V_Float32 T_U_mV_1_1_s16 T_U_mV_256_20_u16 T_U_mV_Float32 T_V_l_256_1_s16 T_V_l_4096_1_s16 T_V_l_64_1_s16 T_V_l_65535_100_u16 T_V_l_Float32 T_V_ml_128_1_s16 T_V_ml_1_1_s16 T_V_ml_32768_1_s16 T_V_ml_Float32 T_V_ul_32_1_u16 T_V_ul_Float32 T_Vpl_clpkm_512_1_u16 T_Vpl_clpkm_Float32 T_a_kphps_16_1_s16 T_a_kphps_Float32 T_a_mps2_128_1_s16 T_a_mps2_Float32 T_c_MJpkg_256_1_s16 T_c_MJpkg_Float32 T_c_kJpgpK_1024_1_s16 T_c_kJpgpK_Float32 T_c_kJpkgpK_128_1_u16 T_c_kJpkgpK_Float32 T_chrg_Ah_1_1_s16 T_chrg_Ah_1_1_u16 T_chrg_Ah_1_1_u8 T_chrg_Ah_256_1_u16 T_chrg_Ah_4194304_1_s32 T_chrg_Ah_512_1_u16 T_chrg_Ah_8_1_u16 T_chrg_Ah_Float32 T_cmp_NA_100_1_s16 T_cmp_NA_128_1_s16 T_cmp_NA_16_1_s16 T_cmp_NA_32768_1_u16 T_cmp_NA_Float32 T_d2n_rpmps2_4_1_s16 T_d2n_rpmps2_Float32 T_dPct_pctps_16_1_s16 T_dPct_pctps_256_1_s16 T_dPct_pctps_Float32 T_dT_degCps_128_1_s16 T_dT_degCps_Float32 T_dV_lph_1_1_s16 T_dV_lph_Float32 T_dV_lpm_128_1_s16 T_dV_lpm_32_1_s16 T_dV_lpm_Float32 T_dV_lps_1024_1_u16 T_dV_lps_4_1_u16 T_dV_lps_Float32 T_dV_mlps_1024_1_s16 T_dV_mlps_Float32 T_d_BitField16 T_dm_gps_128_1_s16 T_dm_gps_128_1_u16 T_dm_gps_256_1_u16 T_dm_gps_Float32 T_dm_mgps_1_1_s16 T_dm_mgps_Float32 T_dn_rpmps_1_1_s16 T_dn_rpmps_2_1_s16 T_dn_rpmps_Float32 T_dp_Paps_1_1_s16 T_dp_Paps_Float32 T_dp_kPaps_1_1_s16 T_dp_kPaps_8_1_s16 T_dp_kPaps_Float32 T_dphi_degps_128_1_s16 T_dphi_degps_8_1_s16 T_dphi_degps_Float32 T_dr_ps_256_1_s16 T_dr_ps_Float32 T_drho_mgplps_1_2_s16 T_drho_mgplps_Float32 T_e_NA_1_1_u8 T_f_Hz_1_1_u16 T_f_Hz_1_1_u32 T_f_Hz_64_1_u16 T_f_Hz_8_1_s16 T_f_Hz_Float32 T_g_BitField32 T_l_km_16_1_s16 T_l_km_1_1_u16 T_l_km_1_1_u32 T_l_km_Float32 T_l_m_1024_1_s16 T_l_m_16_1_s16 T_l_m_1_1_u32 T_l_m_Float32 T_l_mm_16_1_s16 T_l_mm_1_1_u16 T_l_mm_4096_1_s16 T_l_mm_4_1_u8 T_l_mm_64_1_s16 T_l_mm_Float32 T_m_g_1_1_s16 T_m_g_2048_1_s16 T_m_g_32_1_u16 T_m_g_Float32 T_m_kg_1024_1_s16 T_m_kg_1_1_s16 T_m_kg_1_1_u32 T_m_kg_Float32 T_m_mg_128_1_s16 T_m_mg_32_1_s16 T_m_mg_Float32 T_n_rpm_1_1_s16 T_n_rpm_1_25_u8 T_n_rpm_256_50_u16 T_n_rpm_2_25_u8 T_n_rpm_4_1_u16 T_n_rpm_Float32 T_p_MPa_64_1_s16 T_p_MPa_Float32 T_p_Pa_1_1_s16 T_p_Pa_Float32 T_p_kPa_1_10_u16 T_p_kPa_1_1_s16 T_p_kPa_1_1_u8 T_p_kPa_256_1_u16 T_p_kPa_32_1_u16 T_p_kPa_64_1_s16 T_p_kPa_Float32 T_phi_deg_100_1_s16 T_phi_deg_1024_1_s16 T_phi_deg_128_1_s16 T_phi_deg_1_1_u8 T_phi_deg_256_1_s16 T_phi_deg_2_1_s8 T_phi_deg_32_1_s16 T_phi_deg_512_6_s32 T_phi_deg_Float32 T_phi_rad_2048_1_s16 T_phi_rad_Float32 T_r_NA_1024_1_s16 T_r_NA_1024_1_u16 T_r_NA_16384_1_s16 T_r_NA_16_1_s16 T_r_NA_256_1_s8 T_r_NA_256_1_u16 T_r_NA_32768_1_u16 T_r_NA_32_1_u16 T_r_NA_4096_1_s16 T_r_NA_65535_2_u16 T_r_NA_8192_1_u16 T_r_NA_Float32 T_rho_gpl_8192_1_s16 T_rho_gpl_Float32 T_rho_kgpm3_16_1_s16 T_rho_kgpm3_Float32 T_rho_mgpl_1_1_s16 T_rho_mgpl_64_1_s16 T_rho_mgpl_Float32 T_t_hour_1_1_s16 T_t_hour_Float32 T_t_m_1_1_u16 T_t_m_Float32 T_t_ms_1_1_s16 T_t_ms_1_1_u16 T_t_ms_1_1_u32 T_t_ms_4096_1_s16 T_t_ms_64_1_s16 T_t_ms_Float32 T_t_s_1000_1_s16 T_t_s_100_1_s16 T_t_s_10_1_s16 T_t_s_10_1_u16 T_t_s_1_1_s16 T_t_s_1_1_u16 T_t_s_1_1_u32 T_t_s_Float32 T_t_us_10_1_u32 T_t_us_1_1_s16 T_t_us_1_1_u32 T_t_us_1_4_u16 T_t_us_Float32 T_v_kph_1_1_u8 T_v_kph_64_1_s16 T_v_kph_64_1_u16 T_v_kph_Float32 T_v_mps_256_1_s16 T_v_mps_Float32 T_w_radps_32_1_s16 T_w_radps_Float32 T_y_BitField8 T_y_BitFieldDiagProgress T_y_BitFieldDiagStatus T_y_NA_1_1_u8 SInt16 SInt32 SInt8 T_BOOLEAN UInt16 UInt32 UInt8 s16 s32 s8 u16 u32 u8
settings Model: Creator=gaohang  LastModifiedBy=gaohang
settings OptimizationCC: DefaultParameterBehavior=Inlined  UseDivisionForNetSlopeComputation=on  UseFloatMulNetSlope=on  DefaultUnderspecifiedDataType=single  UseSpecifiedMinMax=on  InlineInvariantSignals=on  PassReuseOutputArgsAs=Individual arguments  ZeroExternalMemoryAtStartup=off  ZeroInternalMemoryAtStartup=off  NoFixptDivByZeroProtection=on  EfficientFloat2IntCast=on  LifeSpan=inf  OptimizeBlockOrder=speed  DifferentSizesBufferReuse=on
settings DebuggingCC: SignalInfNanChecking=error  ReadBeforeWriteMsg=EnableAllAsError  WriteAfterWriteMsg=EnableAllAsError  WriteAfterReadMsg=EnableAllAsError  IntegerOverflowMsg=error  ParameterTunabilityLossMsg=error  UniqueDataStoreMsg=error  AssertControl=DisableAll  NonBusSignalsTreatedAsBus=error  SFInvalidInputDataAccessInChartInitDiag=error  SFTransitionOutsideNaturalParentDiag=error  SFUnreachableExecutionPathDiag=error  SFUndirectedBroadcastEventsDiag=error  IntegerSaturationMsg=error
settings HardwareCC: ProdLongLongMode=on
settings ModelReferenceCC: UpdateModelReferenceTargets=IfOutOfDate
settings SFSimCC: SFSimEcho=off  CompileTimeRecursionLimit=0  EnableRuntimeRecursion=off  MATLABDynamicMemAlloc=off
settings RTWCC: SystemTargetFile=autosar.tlc  GenCodeOnly=on  TemplateMakefile=ert_default_tmf  Description=AUTOSAR  GenerateReport=on  BuildConfiguration=Faster Runs  IncludeHyperlinkInReport=on  LaunchReport=on  GenerateTraceInfo=on  GenerateTraceReport=on  GenerateTraceReportSl=on  GenerateTraceReportSf=on  GenerateTraceReportEml=on  GenerateCodeMetricsReport=on
settings CodeAppCC: ForceParamTrailComments=on  IgnoreCustomStorageClasses=off  OperatorAnnotations=on  SimulinkDataObjDesc=on  SFDataObjDesc=on  MATLABFcnDesc=on  InsertBlockDesc=on  StateflowObjectComments=on  MATLABSourceComments=on  EnableCustomComments=on  ReqsInCode=on
settings STFCustomTargetCC: TargetLangStandard=C99 (ISO)  UtilityFuncGeneration=Shared location  MultiwordLength=256  ParMdlRefBuildCompliant=on  CompOptLevelCompliant=on  IncludeMdlTerminateFcn=off  CombineOutputUpdateFcns=on  CombineSignalStateStructs=on  SuppressErrorStatus=on  ERTCustomFileBanners=on  SupportNonFinite=off  SupportComplex=off  SupportContinuousTime=off  SupportNonInlinedSFcns=off  RemoveResetFunc=on  ParenthesesLevel=Maximum  CastingMode=Standards  MATLABClassNameForMDSCustomization=Simulink.SoftwareTarget.ERTCustomization  AutosarCompliant=on  UseToolchainInfoCompliant=on  GenerateSharedConstants=off  LookupTableObjectStructAxisOrder=2,1,3,4,...  LUTObjectStructOrderEvenSpacing=Size,Table,Breakpoints  SystemTargetFile=autosar.tlc
settings ERTTargetCC: TargetLangStandard=C99 (ISO)  UtilityFuncGeneration=Shared location  ConcurrentExecutionCompliant=off  IncludeMdlTerminateFcn=off  CombineSignalStateStructs=on  SuppressErrorStatus=on  SupportNonFinite=off  SupportComplex=off  ParenthesesLevel=Maximum  CastingMode=Standards  ModelStepFunctionPrototypeControlCompliant=off  CPPClassGenCompliant=off  AutosarCompliant=on  GenerateSharedConstants=off  LookupTableObjectStructAxisOrder=2,1,3,4,...  LUTObjectStructOrderEvenSpacing=Size,Table,Breakpoints  GenerateASAP2=on  InlinedParameterPlacement=NonHierarchical  ERTCustomFileTemplate=example_file_process.tlc  EnableSignedLeftShifts=off  EnableSignedRightShifts=off

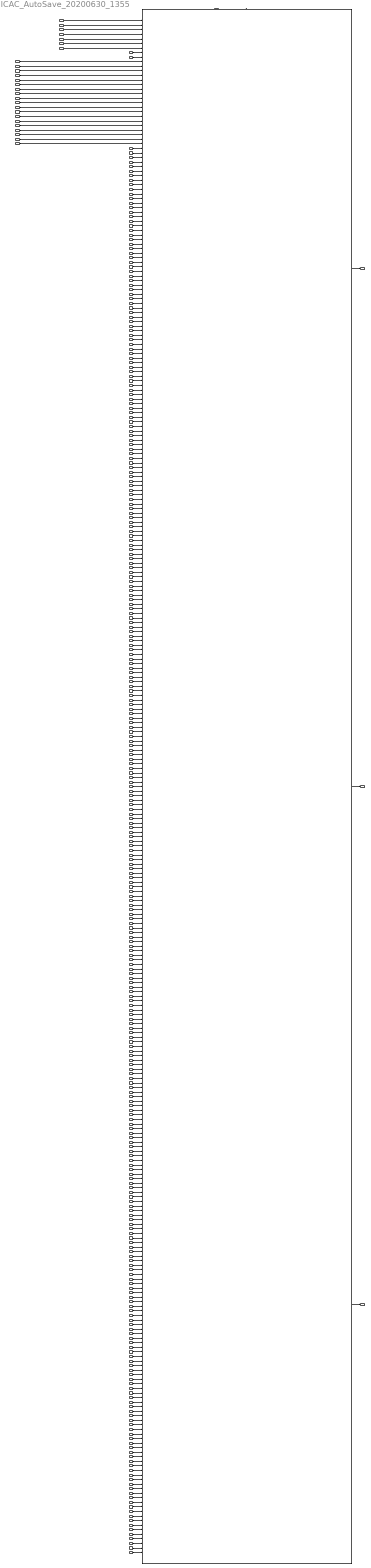
== system ICAC_AutoSave_20200630_1355 ==
  Runnable_ICAC_Step : Inport  SampleTime=0.01  OutputFunctionCall=on
  System_Clock : Inport  Port=2  OutDataTypeStr=UInt16
  ICABva_g_VehParameter : Inport  Port=3  OutDataTypeStr=T_M_Nm_Float32  PortDimensions=60
  ICABva_g_FilterInfo : Inport  Port=4  OutDataTypeStr=T_M_Nm_Float32  PortDimensions=50
  ICABve_d_SignalTStamp : Inport  Port=5  OutDataTypeStr=UInt16
  ICAPva_g_PathPoints : Inport  Port=6  OutDataTypeStr=T_M_Nm_Float32  PortDimensions=1600
  ICAPve_d_PathPointNum : Inport  Port=7  OutDataTypeStr=UInt16
  ICAPve_d_PathValid : Inport  Port=8  OutDataTypeStr=UInt16
  ICAPve_d_SignalTStamp : Inport  Port=9  OutDataTypeStr=UInt16
  ICASva_g_TrajectoryPoints : Inport  Port=10  OutDataTypeStr=T_M_Nm_Float32  PortDimensions=1600
  ICASve_d_TrajectoryPointNum : Inport  Port=11  OutDataTypeStr=UInt16
  ICASve_d_TrajectoryValid : Inport  Port=12  OutDataTypeStr=UInt16
  ICASva_d_TrajectoryPlanState : Inport  Port=13  OutDataTypeStr=UInt16  PortDimensions=10
  ICASve_g_ExpLonAcc : Inport  Port=14  OutDataTypeStr=T_M_Nm_Float32
  ICASve_d_SignalTStamp : Inport  Port=15  OutDataTypeStr=UInt16
  IMAPve_d_EPS_LKA_State : Inport  Port=16  OutDataTypeStr=UInt16
  IMAPve_g_EPS_SW_Trq : Inport  Port=17  OutDataTypeStr=T_M_Nm_Float32
  IMAPve_d_EPS_Error_State : Inport  Port=18  OutDataTypeStr=UInt16
  IMAPve_d_EPS_Trq_State : Inport  Port=19  OutDataTypeStr=UInt16
  IMAPve_d_SAS_Clb_State : Inport  Port=20  OutDataTypeStr=UInt16
  IMAPve_d_SAS_Trim_State : Inport  Port=21  OutDataTypeStr=UInt16
  IMAPve_d_EPS_TrqLim_State : Inport  Port=22  OutDataTypeStr=UInt16
  IMAPve_g_EPS_LKA_Current : Inport  Port=23  OutDataTypeStr=T_M_Nm_Float32
  IMAPve_g_ESC_LatAcc : Inport  Port=24  OutDataTypeStr=T_M_Nm_Float32
  IMAPve_d_ESC_LatAcc_Valid : Inport  Port=25  OutDataTypeStr=UInt16
  IMAPve_g_ESC_YawRate : Inport  Port=26  OutDataTypeStr=T_M_Nm_Float32
  IMAPve_d_ESC_YawRate_Valid : Inport  Port=27  OutDataTypeStr=UInt16
  IMAPve_g_ESC_UnYawRate : Inport  Port=28  OutDataTypeStr=T_M_Nm_Float32
  IMAPve_g_ESC_VehSpd : Inport  Port=29  OutDataTypeStr=T_M_Nm_Float32
  IMAPve_g_ESC_LonAcc : Inport  Port=30  OutDataTypeStr=T_M_Nm_Float32
  IMAPve_d_ESC_LonAcc_Valid : Inport  Port=31  OutDataTypeStr=UInt16
  IMAPve_g_ESC_Brake_Press : Inport  Port=32  OutDataTypeStr=T_M_Nm_Float32
  IMAPve_g_ESC_Static_Slope : Inport  Port=33  OutDataTypeStr=T_M_Nm_Float32
  IMAPve_g_ESC_DySlope_Accuracy : Inport  Port=34  OutDataTypeStr=T_M_Nm_Float32
  IMAPve_g_ESC_DySlope : Inport  Port=35  OutDataTypeStr=T_M_Nm_Float32
  IMAPve_g_SW_Angle : Inport  Port=36  OutDataTypeStr=T_M_Nm_Float32
  IMAPve_g_SW_Angle_Speed : Inport  Port=37  OutDataTypeStr=T_M_Nm_Float32
  IMAPve_d_BCM_HazardLamp : Inport  Port=38  OutDataTypeStr=UInt16
  IMAPve_d_BCM_Left_Light : Inport  Port=39  OutDataTypeStr=UInt16
  IMAPve_d_BCM_Right_Light : Inport  Port=40  OutDataTypeStr=UInt16
  IMAPve_d_ESC_BrakeLamp_Req : Inport  Port=41  OutDataTypeStr=UInt16
  IMAPve_d_BCM_Opening_State : Inport  Port=42  OutDataTypeStr=UInt16
  IMAPve_d_BCM_Trunk_State : Inport  Port=43  OutDataTypeStr=UInt16
  IMAPve_d_BCM_LF_Door_State : Inport  Port=44  OutDataTypeStr=UInt16
  IMAPve_d_BCM_RF_Door_State : Inport  Port=45  OutDataTypeStr=UInt16
  IMAPve_d_BCM_RR_Door_State : Inport  Port=46  OutDataTypeStr=UInt16
  IMAPve_d_BCM_LR_Door_State : Inport  Port=47  OutDataTypeStr=UInt16
  IMAPve_d_SCC_Left_SwitchSig : Inport  Port=48  OutDataTypeStr=UInt16
  IMAPve_d_SCC_Right_SwitchSig : Inport  Port=49  OutDataTypeStr=UInt16
  IMAPve_d_PEPS_Door_Lock_Req : Inport  Port=50  OutDataTypeStr=UInt16
  IMAPve_d_BCM_Door_Lock_State : Inport  Port=51  OutDataTypeStr=UInt16
  IMAPve_d_EMS_ACC_Status : Inport  Port=52  OutDataTypeStr=UInt16
  IMAPve_g_EMS_Pot_WhlT_Max : Inport  Port=53  OutDataTypeStr=T_M_Nm_Float32
  IMAPve_g_EMS_Pot_WhlT_Min : Inport  Port=54  OutDataTypeStr=T_M_Nm_Float32
  IMAPve_g_EMS_RealPedal : Inport  Port=55  OutDataTypeStr=T_M_Nm_Float32
  IMAPve_g_EMS_MaxTWhl : Inport  Port=56  OutDataTypeStr=T_M_Nm_Float32
  IMAPve_g_EMS_MaxTWhl_Offset : Inport  Port=57  OutDataTypeStr=T_M_Nm_Float32
  IMAPve_g_EMS_MinTWhl : Inport  Port=58  OutDataTypeStr=T_M_Nm_Float32
  IMAPve_g_EMS_MinTWhl_Offset : Inport  Port=59  OutDataTypeStr=T_M_Nm_Float32
  IMAPve_g_EMS_Actual_FlwT : Inport  Port=60  OutDataTypeStr=T_M_Nm_Float32
  IMAPve_g_EMS_Actual_IndT : Inport  Port=61  OutDataTypeStr=T_M_Nm_Float32
  IMAPve_g_EMS_Realize_TWhl : Inport  Port=62  OutDataTypeStr=T_M_Nm_Float32
  IMAPve_g_EMS_ACC_VirtualPedal : Inport  Port=63  OutDataTypeStr=T_M_Nm_Float32
  IMAPve_d_EMS_AccPedal_Fault : Inport  Port=64  OutDataTypeStr=UInt16
  IMAPve_g_EMS_Driver_Torque : Inport  Port=65  OutDataTypeStr=T_M_Nm_Float32
  IMAPve_d_ESC_Brake_Effort : Inport  Port=66  OutDataTypeStr=UInt16
  IMAPve_g_EMS_Engine_Speed : Inport  Port=67  OutDataTypeStr=T_M_Nm_Float32
  IMAPve_d_ESC_Veh_Standstill : Inport  Port=68  OutDataTypeStr=UInt16
  IMAPve_d_TCU_Actual_Gear : Inport  Port=69  OutDataTypeStr=UInt16
  IMAPve_d_TCU_Target_Gear : Inport  Port=70  OutDataTypeStr=UInt16
  IMAPve_d_TCU_PRND_State : Inport  Port=71  OutDataTypeStr=UInt16
  IMAPve_d_BCM_Ignition_State : Inport  Port=72  OutDataTypeStr=UInt16
  IMAPve_d_ACU_Driver_Belt : Inport  Port=73  OutDataTypeStr=UInt16
  IMAPve_d_SWS_Fault_Code : Inport  Port=74  OutDataTypeStr=UInt16
  IMAPve_d_SWS_Failure_Status : Inport  Port=75  OutDataTypeStr=UInt16
  IMAPve_d_ESC_OFF : Inport  Port=76  OutDataTypeStr=UInt16
  IMAPve_d_ESC_AlarmSig : Inport  Port=77  OutDataTypeStr=UInt16
  IMAPve_d_Speed_Limit_Switch : Inport  Port=78  OutDataTypeStr=UInt16
  IMAPve_d_ESC_ESC_Active : Inport  Port=79  OutDataTypeStr=UInt16
  IMAPve_d_ESC_MSR_Active : Inport  Port=80  OutDataTypeStr=UInt16
  IMAPve_d_ESC_TCS_Active : Inport  Port=81  OutDataTypeStr=UInt16
  IMAPve_d_ESC_VehSpd_Valid : Inport  Port=82  OutDataTypeStr=UInt16
  IMAPve_d_Brake_Pedal_Fault : Inport  Port=83  OutDataTypeStr=UInt16
  IMAPve_d_ESC_ABS_Active : Inport  Port=84  OutDataTypeStr=UInt16
  IMAPve_d_ESC_ABS_Valid : Inport  Port=85  OutDataTypeStr=UInt16
  IMAPve_d_ESC_ABS_AlarmSig : Inport  Port=86  OutDataTypeStr=UInt16
  IMAPve_d_ESC_FL_WheelPulVal : Inport  Port=87  OutDataTypeStr=UInt16
  IMAPve_d_ESC_FR_WheelPulVal : Inport  Port=88  OutDataTypeStr=UInt16
  IMAPve_d_ESC_RL_WheelPulVal : Inport  Port=89  OutDataTypeStr=UInt16
  IMAPve_d_ESC_RR_WheelPulVal : Inport  Port=90  OutDataTypeStr=UInt16
  IMAPve_g_ESC_FL_WhlSpd : Inport  Port=91  OutDataTypeStr=T_M_Nm_Float32
  IMAPve_d_ESC_FL_WhlSpd_Fault : Inport  Port=92  OutDataTypeStr=UInt16
  IMAPve_g_ESC_FR_WhlSpd : Inport  Port=93  OutDataTypeStr=T_M_Nm_Float32
  IMAPve_d_ESC_FR_WhlSpd_Fault : Inport  Port=94  OutDataTypeStr=UInt16
  IMAPve_g_ESC_RL_WhlSpd : Inport  Port=95  OutDataTypeStr=T_M_Nm_Float32
  IMAPve_d_ESC_RL_WhlSpd_Fault : Inport  Port=96  OutDataTypeStr=UInt16
  IMAPve_g_ESC_RR_WhlSpd : Inport  Port=97  OutDataTypeStr=T_M_Nm_Float32
  IMAPve_d_ESC_RR_WhlSpd_Fault : Inport  Port=98  OutDataTypeStr=UInt16
  IMAPve_d_ESC_FL_Wheel_Pulse : Inport  Port=99  OutDataTypeStr=UInt16
  IMAPve_d_ESC_FR_Wheel_Pulse : Inport  Port=100  OutDataTypeStr=UInt16
  IMAPve_d_ESC_RL_Wheel_Pulse : Inport  Port=101  OutDataTypeStr=UInt16
  IMAPve_d_ESC_RR_Wheel_Pulse : Inport  Port=102  OutDataTypeStr=UInt16
  IMAPve_d_TCU_AT_Failure : Inport  Port=103  OutDataTypeStr=UInt16
  IMAPve_d_TCU_Shift_Valid : Inport  Port=104  OutDataTypeStr=UInt16
  IMAPve_d_TCU_DCT_Clutch_State : Inport  Port=105  OutDataTypeStr=UInt16
  IMAPve_d_TCU_Gear_Engage : Inport  Port=106  OutDataTypeStr=UInt16
  IMAPve_d_TCU_Select_ATMode : Inport  Port=107  OutDataTypeStr=UInt16
  IMAPve_d_EMS_Engine_Status : Inport  Port=108  OutDataTypeStr=UInt16
  IMAPve_d_EMS_Gearbox_CtlAvail : Inport  Port=109  OutDataTypeStr=UInt16
  IMAPve_d_ESC_Brake_Failsafe : Inport  Port=110  OutDataTypeStr=UInt16
  IMAPve_d_ESC_AEB_Status : Inport  Port=111  OutDataTypeStr=UInt16
  IMAPve_d_ESC_AEB_Available : Inport  Port=112  OutDataTypeStr=UInt16
  IMAPve_d_ESC_AEB_Active : Inport  Port=113  OutDataTypeStr=UInt16
  IMAPve_d_ESC_ACC_Status : Inport  Port=114  OutDataTypeStr=UInt16
  IMAPve_d_ESC_ACC_Available : Inport  Port=115  OutDataTypeStr=UInt16
  IMAPve_d_ESC_ACC_Active : Inport  Port=116  OutDataTypeStr=UInt16
  IMAPve_d_EMS_ACC_Effective : Inport  Port=117  OutDataTypeStr=UInt16
  IMAPve_d_BCM_FrontWiper_State : Inport  Port=118  OutDataTypeStr=UInt16
  IMAPve_d_BCM_CHMSL_Status : Inport  Port=119  OutDataTypeStr=UInt16
  IMAPve_d_BCM_BrakeLamp_State : Inport  Port=120  OutDataTypeStr=UInt16
  IMAPve_d_GW_Brake_Only_Req : Inport  Port=121  OutDataTypeStr=UInt16
  IMAPve_d_ACU_Passenger_Belt : Inport  Port=122  OutDataTypeStr=UInt16
  IMAPve_d_EMS_ACC_CtlAvail : Inport  Port=123  OutDataTypeStr=UInt16
  IMAPve_d_EMS_ACC_Inhibited : Inport  Port=124  OutDataTypeStr=UInt16
  IMAPve_d_EMS_Brake_Pedal : Inport  Port=125  OutDataTypeStr=UInt16
  IMAPve_d_BCM_LowBeam_State : Inport  Port=126  OutDataTypeStr=UInt16
  IMAPve_d_BCM_HighBeam_State : Inport  Port=127  OutDataTypeStr=UInt16
  IMAPve_d_EPB_Status : Inport  Port=128  OutDataTypeStr=UInt16
  IMAPve_d_EPB_Display_Req : Inport  Port=129  OutDataTypeStr=UInt16
  IMAPve_d_EPB_Warn_Req : Inport  Port=130  OutDataTypeStr=UInt16
  IMAPve_d_EPB_Switch_State : Inport  Port=131  OutDataTypeStr=UInt16
  IMAPve_d_EPB_Switch_Valid : Inport  Port=132  OutDataTypeStr=UInt16
  IMAPve_d_ESC_Drive_Direction : Inport  Port=133  OutDataTypeStr=UInt16
  IMAPve_d_ESC_Hold_State : Inport  Port=134  OutDataTypeStr=UInt16
  IMAPve_d_EPS_Steer_Hold_State : Inport  Port=135  OutDataTypeStr=UInt16
  IMAPve_d_EPS_Warning_State : Inport  Port=136  OutDataTypeStr=UInt16
  IMAPve_g_EPS_PowerCon : Inport  Port=137  OutDataTypeStr=T_M_Nm_Float32
  IMAPve_d_ESC_EBD_AlarmSig : Inport  Port=138  OutDataTypeStr=UInt16
  IMAPve_d_ESC_AVH_Status : Inport  Port=139  OutDataTypeStr=UInt16
  IMAPve_d_Radar_Detective_Req : Inport  Port=140  OutDataTypeStr=UInt16
  IMAPve_g_BCM_Battery_Voltage : Inport  Port=141  OutDataTypeStr=T_M_Nm_Float32
  IMAPve_d_TBOX_LocalTimeY : Inport  Port=142  OutDataTypeStr=UInt16
  IMAPve_d_TBOX_LocalTimeM : Inport  Port=143  OutDataTypeStr=UInt16
  IMAPve_d_TBOX_LocalTimeD : Inport  Port=144  OutDataTypeStr=UInt16
  IMAPve_d_TBOX_LocalTimeH : Inport  Port=145  OutDataTypeStr=UInt16
  IMAPve_d_TBOX_LocalTimeMin : Inport  Port=146  OutDataTypeStr=UInt16
  IMAPve_d_TBOX_LocalTimeS : Inport  Port=147  OutDataTypeStr=UInt16
  IMAPve_d_TBOX_LocalTime_Valid : Inport  Port=148  OutDataTypeStr=UInt16
  IMAPve_d_TPMS_Warn_Indicate : Inport  Port=149  OutDataTypeStr=UInt16
  IMAPve_d_Radar_State : Inport  Port=150  OutDataTypeStr=UInt16
  IMAPve_d_ACC_Desired_Headway : Inport  Port=151  OutDataTypeStr=UInt16
  IMAPve_d_Time_System_Clock : Inport  Port=152  OutDataTypeStr=UInt16
  IMAPve_d_Signal_Time_Stamp : Inport  Port=153  OutDataTypeStr=UInt16
  IMAPve_g_GW_IC_Odometer : Inport  Port=154  OutDataTypeStr=T_M_Nm_Float32
  IMAPve_g_FAPA_State : Inport  Port=155  OutDataTypeStr=T_M_Nm_Float32
  IMAPve_d_Outside_Temp : Inport  Port=156  OutDataTypeStr=UInt16
  IMAPve_d_ORI_CIPV_ID : Inport  Port=157  OutDataTypeStr=UInt16
  IMAPve_d_ORI_Obj_Num : Inport  Port=158  OutDataTypeStr=UInt16
  IMAPva_g_ORI_Probability : Inport  Port=159  OutDataTypeStr=T_M_Nm_Float32  PortDimensions=16
  IMAPva_d_ORI_Obj_Class : Inport  Port=160  OutDataTypeStr=UInt16  PortDimensions=16
  IMAPva_d_ORI_Obj_Motion : Inport  Port=161  OutDataTypeStr=UInt16  PortDimensions=16
  IMAPva_g_ORI_Obj_RelVel : Inport  Port=162  OutDataTypeStr=T_M_Nm_Float32  PortDimensions=16
  IMAPva_g_ORI_Obj_LongDis : Inport  Port=163  OutDataTypeStr=T_M_Nm_Float32  PortDimensions=16
  IMAPva_d_ORI_Obj_Lane : Inport  Port=164  OutDataTypeStr=UInt16  PortDimensions=16
  IMAPva_g_ORI_Obj_LAngle : Inport  Port=165  OutDataTypeStr=T_M_Nm_Float32  PortDimensions=16
  IMAPva_g_ORI_Obj_RAngle : Inport  Port=166  OutDataTypeStr=T_M_Nm_Float32  PortDimensions=16
  IMAPva_g_ORI_Obj_Width : Inport  Port=167  OutDataTypeStr=T_M_Nm_Float32  PortDimensions=16
  IMAPva_d_ORI_Obj_ID : Inport  Port=168  OutDataTypeStr=UInt16  PortDimensions=16
  IMAPve_d_ORI_Lane_Valid : Inport  Port=169  OutDataTypeStr=UInt16
  IMAPve_d_ORI_Lane_ConsArea : Inport  Port=170  OutDataTypeStr=UInt16
  IMAPve_d_ORI_Lane_RoadType : Inport  Port=171  OutDataTypeStr=UInt16
  IMAPve_g_ORI_L0_C3 : Inport  Port=172  OutDataTypeStr=T_M_Nm_Float32
  IMAPve_g_ORI_L0_C2 : Inport  Port=173  OutDataTypeStr=T_M_Nm_Float32
  IMAPve_g_ORI_L0_C1 : Inport  Port=174  OutDataTypeStr=T_M_Nm_Float32
  IMAPve_g_ORI_L0_C0 : Inport  Port=175  OutDataTypeStr=T_M_Nm_Float32
  IMAPve_d_ORI_L0_Q : Inport  Port=176  OutDataTypeStr=UInt16
  IMAPve_d_ORI_L0_Type : Inport  Port=177  OutDataTypeStr=UInt16
  IMAPve_g_ORI_L0_VR : Inport  Port=178  OutDataTypeStr=T_M_Nm_Float32
  IMAPve_g_ORI_L0_TLC : Inport  Port=179  OutDataTypeStr=T_M_Nm_Float32
  IMAPve_g_ORI_L0_W : Inport  Port=180  OutDataTypeStr=T_M_Nm_Float32
  IMAPve_d_ORI_L0_LC : Inport  Port=181  OutDataTypeStr=UInt16
  IMAPve_g_ORI_L1_C3 : Inport  Port=182  OutDataTypeStr=T_M_Nm_Float32
  IMAPve_g_ORI_L1_C2 : Inport  Port=183  OutDataTypeStr=T_M_Nm_Float32
  IMAPve_g_ORI_L1_C1 : Inport  Port=184  OutDataTypeStr=T_M_Nm_Float32
  IMAPve_g_ORI_L1_C0 : Inport  Port=185  OutDataTypeStr=T_M_Nm_Float32
  IMAPve_d_ORI_L1_Q : Inport  Port=186  OutDataTypeStr=UInt16
  IMAPve_d_ORI_L1_Type : Inport  Port=187  OutDataTypeStr=UInt16
  IMAPve_g_ORI_L1_VR : Inport  Port=188  OutDataTypeStr=T_M_Nm_Float32
  IMAPve_g_ORI_L1_TLC : Inport  Port=189  OutDataTypeStr=T_M_Nm_Float32
  IMAPve_g_ORI_L1_W : Inport  Port=190  OutDataTypeStr=T_M_Nm_Float32
  IMAPve_d_ORI_L1_LC : Inport  Port=191  OutDataTypeStr=UInt16
  IMAPve_g_ORI_R0_C3 : Inport  Port=192  OutDataTypeStr=T_M_Nm_Float32
  IMAPve_g_ORI_R0_C2 : Inport  Port=193  OutDataTypeStr=T_M_Nm_Float32
  IMAPve_g_ORI_R0_C1 : Inport  Port=194  OutDataTypeStr=T_M_Nm_Float32
  IMAPve_g_ORI_R0_C0 : Inport  Port=195  OutDataTypeStr=T_M_Nm_Float32
  IMAPve_d_ORI_R0_Q : Inport  Port=196  OutDataTypeStr=UInt16
  IMAPve_d_ORI_R0_LT : Inport  Port=197  OutDataTypeStr=UInt16
  IMAPve_g_ORI_R0_VR : Inport  Port=198  OutDataTypeStr=T_M_Nm_Float32
  IMAPve_g_ORI_R0_TLC : Inport  Port=199  OutDataTypeStr=T_M_Nm_Float32
  IMAPve_g_ORI_R0_W : Inport  Port=200  OutDataTypeStr=T_M_Nm_Float32
  IMAPve_d_ORI_R0_LC : Inport  Port=201  OutDataTypeStr=UInt16
  IMAPve_g_ORI_R1_C3 : Inport  Port=202  OutDataTypeStr=T_M_Nm_Float32
  IMAPve_g_ORI_R1_C2 : Inport  Port=203  OutDataTypeStr=T_M_Nm_Float32
  IMAPve_g_ORI_R1_C1 : Inport  Port=204  OutDataTypeStr=T_M_Nm_Float32
  IMAPve_g_ORI_R1_C0 : Inport  Port=205  OutDataTypeStr=T_M_Nm_Float32
  IMAPve_d_ORI_R1_Q : Inport  Port=206  OutDataTypeStr=UInt16
  IMAPve_d_ORI_R1_LT : Inport  Port=207  OutDataTypeStr=UInt16
  IMAPve_g_ORI_R1_VR : Inport  Port=208  OutDataTypeStr=T_M_Nm_Float32
  IMAPve_g_ORI_R1_TLC : Inport  Port=209  OutDataTypeStr=T_M_Nm_Float32
  IMAPve_g_ORI_R1_W : Inport  Port=210  OutDataTypeStr=T_M_Nm_Float32
  IMAPve_d_ORI_R1_LC : Inport  Port=211  OutDataTypeStr=UInt16
  IMAPve_d_Sensor_Status : Inport  Port=212  OutDataTypeStr=UInt16
  IMAPve_d_LF_Radar_Status : Inport  Port=213  OutDataTypeStr=UInt16
  IMAPve_d_RF_Radar_Status : Inport  Port=214  OutDataTypeStr=UInt16
  IMAPve_d_LR_Radar_Status : Inport  Port=215  OutDataTypeStr=UInt16
  IMAPve_d_RR_Radar_Status : Inport  Port=216  OutDataTypeStr=UInt16
  IMAPve_d_Fusion_Status : Inport  Port=217  OutDataTypeStr=UInt16
  IMAPve_g_Fusion_Time_Stamp : Inport  Port=218  OutDataTypeStr=T_M_Nm_Float32
  IMAPve_d_obj_Num : Inport  Port=219  OutDataTypeStr=UInt16
  IMAPva_d_obj_id : Inport  Port=220  OutDataTypeStr=UInt16  PortDimensions=40
  IMAPva_g_obj_pos_x : Inport  Port=221  OutDataTypeStr=T_M_Nm_Float32  PortDimensions=40
  IMAPva_g_obj_pos_y : Inport  Port=222  OutDataTypeStr=T_M_Nm_Float32  PortDimensions=40
  IMAPva_g_obj_vel_x : Inport  Port=223  OutDataTypeStr=T_M_Nm_Float32  PortDimensions=40
  IMAPva_g_obj_vel_y : Inport  Port=224  OutDataTypeStr=T_M_Nm_Float32  PortDimensions=40
  IMAPva_g_obj_acc_x : Inport  Port=225  OutDataTypeStr=T_M_Nm_Float32  PortDimensions=40
  IMAPva_g_obj_acc_y : Inport  Port=226  OutDataTypeStr=T_M_Nm_Float32  PortDimensions=40
  IMAPva_g_obj_pos_var_x : Inport  Port=227  OutDataTypeStr=T_M_Nm_Float32  PortDimensions=40
  IMAPva_g_obj_pos_var_y : Inport  Port=228  OutDataTypeStr=T_M_Nm_Float32  PortDimensions=40
  IMAPva_g_obj_pos_var_xy : Inport  Port=229  OutDataTypeStr=T_M_Nm_Float32  PortDimensions=40
  IMAPva_g_obj_vel_var_x : Inport  Port=230  OutDataTypeStr=T_M_Nm_Float32  PortDimensions=40
  IMAPva_g_obj_vel_var_y : Inport  Port=231  OutDataTypeStr=T_M_Nm_Float32  PortDimensions=40
  IMAPva_g_obj_vel_var_xy : Inport  Port=232  OutDataTypeStr=T_M_Nm_Float32  PortDimensions=40
  IMAPva_g_obj_width : Inport  Port=233  OutDataTypeStr=T_M_Nm_Float32  PortDimensions=40
  IMAPva_g_obj_length : Inport  Port=234  OutDataTypeStr=T_M_Nm_Float32  PortDimensions=40
  IMAPva_d_obj_fusion_type : Inport  Port=235  OutDataTypeStr=UInt16  PortDimensions=40
  IMAPva_d_obj_class : Inport  Port=236  OutDataTypeStr=UInt16  PortDimensions=40
  IMAPva_d_obj_lane : Inport  Port=237  OutDataTypeStr=UInt16  PortDimensions=40
  IMAPva_d_obj_status : Inport  Port=238  OutDataTypeStr=UInt16  PortDimensions=40
  IMAPva_d_obj_cam_asso_id : Inport  Port=239  OutDataTypeStr=UInt16  PortDimensions=40
  IMAPva_g_obj_con : Inport  Port=240  OutDataTypeStr=T_M_Nm_Float32  PortDimensions=40
  IMAPva_g_obj_age : Inport  Port=241  OutDataTypeStr=T_M_Nm_Float32  PortDimensions=40
  IMAPva_d_obj_TurnLight : Inport  Port=242  OutDataTypeStr=UInt16  PortDimensions=40
  IMAPva_d_obj_BrakeLight : Inport  Port=243  OutDataTypeStr=UInt16  PortDimensions=40
  IMAPva_d_obj_MotionStatus : Inport  Port=244  OutDataTypeStr=UInt16  PortDimensions=40
  IMAPva_d_obj_ACC : Inport  Port=245  OutDataTypeStr=UInt16  PortDimensions=40
  IMAPva_d_obj_AEB : Inport  Port=246  OutDataTypeStr=UInt16  PortDimensions=40
  IMAPva_d_obj_ELK : Inport  Port=247  OutDataTypeStr=UInt16  PortDimensions=40
  IMAPva_d_obj_ALC : Inport  Port=248  OutDataTypeStr=UInt16  PortDimensions=40
  IMAPva_d_obj_ESA : Inport  Port=249  OutDataTypeStr=UInt16  PortDimensions=40
  IMAPva_d_obj_JA : Inport  Port=250  OutDataTypeStr=UInt16  PortDimensions=40
  IMAPve_d_Lane_Valid : Inport  Port=251  OutDataTypeStr=UInt16
  IMAPve_d_Road_Type : Inport  Port=252  OutDataTypeStr=UInt16
  IMAPve_d_ConsArea : Inport  Port=253  OutDataTypeStr=UInt16
  IMAPve_g_L0_C0 : Inport  Port=254  OutDataTypeStr=T_M_Nm_Float32
  IMAPve_g_L0_C1 : Inport  Port=255  OutDataTypeStr=T_M_Nm_Float32
  IMAPve_g_L0_C2 : Inport  Port=256  OutDataTypeStr=T_M_Nm_Float32
  IMAPve_g_L0_C3 : Inport  Port=257  OutDataTypeStr=T_M_Nm_Float32
  IMAPve_g_L0_VR : Inport  Port=258  OutDataTypeStr=T_M_Nm_Float32
  IMAPve_d_L0_Q : Inport  Port=259  OutDataTypeStr=UInt16
  IMAPve_d_L0_Type : Inport  Port=260  OutDataTypeStr=UInt16
  IMAPve_g_L0_Confidence : Inport  Port=261  OutDataTypeStr=T_M_Nm_Float32
  IMAPve_g_L0_W : Inport  Port=262  OutDataTypeStr=T_M_Nm_Float32
  IMAPve_g_L0_TLC : Inport  Port=263  OutDataTypeStr=T_M_Nm_Float32
  IMAPve_d_L0_LC : Inport  Port=264  OutDataTypeStr=UInt16
  IMAPve_g_R0_C0 : Inport  Port=265  OutDataTypeStr=T_M_Nm_Float32
  IMAPve_g_R0_C1 : Inport  Port=266  OutDataTypeStr=T_M_Nm_Float32
  IMAPve_g_R0_C2 : Inport  Port=267  OutDataTypeStr=T_M_Nm_Float32
  IMAPve_g_R0_C3 : Inport  Port=268  OutDataTypeStr=T_M_Nm_Float32
  IMAPve_g_R0_VR : Inport  Port=269  OutDataTypeStr=T_M_Nm_Float32
  IMAPve_d_R0_Q : Inport  Port=270  OutDataTypeStr=UInt16
  IMAPve_d_R0_Type : Inport  Port=271  OutDataTypeStr=UInt16
  IMAPve_g_R0_Confidence : Inport  Port=272  OutDataTypeStr=T_M_Nm_Float32
  IMAPve_g_R0_W : Inport  Port=273  OutDataTypeStr=T_M_Nm_Float32
  IMAPve_g_R0_TLC : Inport  Port=274  OutDataTypeStr=T_M_Nm_Float32
  IMAPve_d_R0_LC : Inport  Port=275  OutDataTypeStr=UInt16
  IMAPve_g_L1_C0 : Inport  Port=276  OutDataTypeStr=T_M_Nm_Float32
  IMAPve_g_L1_C1 : Inport  Port=277  OutDataTypeStr=T_M_Nm_Float32
  IMAPve_g_L1_C2 : Inport  Port=278  OutDataTypeStr=T_M_Nm_Float32
  IMAPve_g_L1_C3 : Inport  Port=279  OutDataTypeStr=T_M_Nm_Float32
  IMAPve_g_L1_VR : Inport  Port=280  OutDataTypeStr=T_M_Nm_Float32
  IMAPve_d_L1_Q : Inport  Port=281  OutDataTypeStr=UInt16
  IMAPve_d_L1_Type : Inport  Port=282  OutDataTypeStr=UInt16
  IMAPve_g_L1_Confidence : Inport  Port=283  OutDataTypeStr=T_M_Nm_Float32
  IMAPve_g_L1_W : Inport  Port=284  OutDataTypeStr=T_M_Nm_Float32
  IMAPve_g_L1_TLC : Inport  Port=285  OutDataTypeStr=T_M_Nm_Float32
  IMAPve_d_L1_LC : Inport  Port=286  OutDataTypeStr=UInt16
  IMAPve_g_R1_C0 : Inport  Port=287  OutDataTypeStr=T_M_Nm_Float32
  IMAPve_g_R1_C1 : Inport  Port=288  OutDataTypeStr=T_M_Nm_Float32
  IMAPve_g_R1_C2 : Inport  Port=289  OutDataTypeStr=T_M_Nm_Float32
  IMAPve_g_R1_C3 : Inport  Port=290  OutDataTypeStr=T_M_Nm_Float32
  IMAPve_g_R1_VR : Inport  Port=291  OutDataTypeStr=T_M_Nm_Float32
  IMAPve_d_R1_Q : Inport  Port=292  OutDataTypeStr=UInt16
  IMAPve_d_R1_Type : Inport  Port=293  OutDataTypeStr=UInt16
  IMAPve_g_R1_Confidence : Inport  Port=294  OutDataTypeStr=T_M_Nm_Float32
  IMAPve_g_R1_W : Inport  Port=295  OutDataTypeStr=T_M_Nm_Float32
  IMAPve_g_R1_TLC : Inport  Port=296  OutDataTypeStr=T_M_Nm_Float32
  IMAPve_d_R1_LC : Inport  Port=297  OutDataTypeStr=UInt16
  IMAPve_g_L0_C0_Back : Inport  Port=298  OutDataTypeStr=T_M_Nm_Float32
  IMAPve_g_L0_C1_Back : Inport  Port=299  OutDataTypeStr=T_M_Nm_Float32
  IMAPve_g_L0_C2_Back : Inport  Port=300  OutDataTypeStr=T_M_Nm_Float32
  IMAPve_g_L0_C3_Back : Inport  Port=301  OutDataTypeStr=T_M_Nm_Float32
  IMAPve_g_L0_Range_Back : Inport  Port=302  OutDataTypeStr=T_M_Nm_Float32
  IMAPve_g_L0_C0_FR_Pred : Inport  Port=303  OutDataTypeStr=T_M_Nm_Float32
  IMAPve_g_L0_C1_FR_Pred : Inport  Port=304  OutDataTypeStr=T_M_Nm_Float32
  IMAPve_g_L0_C2_FR_Pred : Inport  Port=305  OutDataTypeStr=T_M_Nm_Float32
  IMAPve_g_L0_Range_FR_Pred : Inport  Port=306  OutDataTypeStr=T_M_Nm_Float32
  IMAPve_g_R0_C0_Back : Inport  Port=307  OutDataTypeStr=T_M_Nm_Float32
  IMAPve_g_R0_C1_Back : Inport  Port=308  OutDataTypeStr=T_M_Nm_Float32
  IMAPve_g_R0_C2_Back : Inport  Port=309  OutDataTypeStr=T_M_Nm_Float32
  IMAPve_g_R0_C3_Back : Inport  Port=310  OutDataTypeStr=T_M_Nm_Float32
  IMAPve_g_R0_Range_Back : Inport  Port=311  OutDataTypeStr=T_M_Nm_Float32
  IMAPve_g_R0_C0_FR_Pred : Inport  Port=312  OutDataTypeStr=T_M_Nm_Float32
  IMAPve_g_R0_C1_FR_Pred : Inport  Port=313  OutDataTypeStr=T_M_Nm_Float32
  IMAPve_g_R0_C2_FR_Pred : Inport  Port=314  OutDataTypeStr=T_M_Nm_Float32
  IMAPve_g_R0_Range_FR_Pred : Inport  Port=315  OutDataTypeStr=T_M_Nm_Float32
  IMAPve_g_L1_C0_Back : Inport  Port=316  OutDataTypeStr=T_M_Nm_Float32
  IMAPve_g_L1_C1_Back : Inport  Port=317  OutDataTypeStr=T_M_Nm_Float32
  IMAPve_g_L1_C2_Back : Inport  Port=318  OutDataTypeStr=T_M_Nm_Float32
  IMAPve_g_L1_C3_Back : Inport  Port=319  OutDataTypeStr=T_M_Nm_Float32
  IMAPve_g_L1_Range_Back : Inport  Port=320  OutDataTypeStr=T_M_Nm_Float32
  IMAPve_g_L1_C0_FR_Pred : Inport  Port=321  OutDataTypeStr=T_M_Nm_Float32
  IMAPve_g_L1_C1_FR_Pred : Inport  Port=322  OutDataTypeStr=T_M_Nm_Float32
  IMAPve_g_L1_C2_FR_Pred : Inport  Port=323  OutDataTypeStr=T_M_Nm_Float32
  IMAPve_g_L1_Range_FR_Pred : Inport  Port=324  OutDataTypeStr=T_M_Nm_Float32
  IMAPve_g_R1_C0_Back : Inport  Port=325  OutDataTypeStr=T_M_Nm_Float32
  IMAPve_g_R1_C1_Back : Inport  Port=326  OutDataTypeStr=T_M_Nm_Float32
  IMAPve_g_R1_C2_Back : Inport  Port=327  OutDataTypeStr=T_M_Nm_Float32
  IMAPve_g_R1_C3_Back : Inport  Port=328  OutDataTypeStr=T_M_Nm_Float32
  IMAPve_g_R1_Range_Back : Inport  Port=329  OutDataTypeStr=T_M_Nm_Float32
  IMAPve_g_R1_C0_FR_Pred : Inport  Port=330  OutDataTypeStr=T_M_Nm_Float32
  IMAPve_g_R1_C1_FR_Pred : Inport  Port=331  OutDataTypeStr=T_M_Nm_Float32
  IMAPve_g_R1_C2_FR_Pred : Inport  Port=332  OutDataTypeStr=T_M_Nm_Float32
  IMAPve_g_R1_Range_FR_Pred : Inport  Port=333  OutDataTypeStr=T_M_Nm_Float32
  IMAPve_d_Sign_ISA_Value : Inport  Port=334  OutDataTypeStr=UInt16
  IMAPve_d_TSR_Sign_Type : Inport  Port=335  OutDataTypeStr=UInt16
  IMAPve_d_Camera_Signal_Fault : Inport  Port=336  OutDataTypeStr=UInt16
  IMAPve_d_Radar_Status : Inport  Port=337  OutDataTypeStr=UInt16
  IMAPve_d_Camera_Status : Inport  Port=338  OutDataTypeStr=UInt16
  ICAC : Subsystem  TreatAsAtomicUnit=on
  ICACve_g_SteerAngleCmd : Outport  OutDataTypeStr=T_M_Nm_Float32
  ICACve_d_SteerAngleVld : Outport  Port=2  OutDataTypeStr=UInt16
  ICACve_d_SignalTStamp : Outport  Port=3  OutDataTypeStr=UInt16
  wires:
  System_Clock/1 -> ICAC/1(System_Clock)
  ICABva_g_VehParameter/1 -> ICAC/2(ICABva_g_VehParameter)
  ICABva_g_FilterInfo/1 -> ICAC/3(ICABva_g_FilterInfo)
  ICABve_d_SignalTStamp/1 -> ICAC/4(ICABve_d_SignalTStamp)
  ICAPva_g_PathPoints/1 -> ICAC/5(ICAPva_g_PathPoints)
  ICAPve_d_PathPointNum/1 -> ICAC/6(ICAPve_d_PathPointNum)
  ICAPve_d_PathValid/1 -> ICAC/7(ICAPve_d_PathValid)
  ICAPve_d_SignalTStamp/1 -> ICAC/8(ICAPve_d_SignalTStamp)
  ICASva_g_TrajectoryPoints/1 -> ICAC/9(ICASva_g_TrajectoryPoints)
  ICASve_d_TrajectoryPointNum/1 -> ICAC/10(ICASve_d_TrajectoryPointNum)
  ICASve_d_TrajectoryValid/1 -> ICAC/11(ICASve_d_TrajectoryValid)
  ICASva_d_TrajectoryPlanState/1 -> ICAC/12(ICASva_d_TrajectoryPlanState)
  ICASve_g_ExpLonAcc/1 -> ICAC/13(ICASve_g_ExpLonAcc)
  ICASve_d_SignalTStamp/1 -> ICAC/14(ICASve_d_SignalTStamp)
  IMAPve_d_EPS_LKA_State/1 -> ICAC/15(IMAPve_d_EPS_LKA_State)
  IMAPve_g_EPS_SW_Trq/1 -> ICAC/16(IMAPve_g_EPS_SW_Trq)
  IMAPve_d_EPS_Error_State/1 -> ICAC/17(IMAPve_d_EPS_Error_State)
  IMAPve_d_EPS_Trq_State/1 -> ICAC/18(IMAPve_d_EPS_Trq_State)
  IMAPve_d_SAS_Clb_State/1 -> ICAC/19(IMAPve_d_SAS_Clb_State)
  IMAPve_d_SAS_Trim_State/1 -> ICAC/20(IMAPve_d_SAS_Trim_State)
  IMAPve_d_EPS_TrqLim_State/1 -> ICAC/21(IMAPve_d_EPS_TrqLim_State)
  IMAPve_g_EPS_LKA_Current/1 -> ICAC/22(IMAPve_g_EPS_LKA_Current)
  IMAPve_g_ESC_LatAcc/1 -> ICAC/23(IMAPve_g_ESC_LatAcc)
  IMAPve_d_ESC_LatAcc_Valid/1 -> ICAC/24(IMAPve_d_ESC_LatAcc_Valid)
  IMAPve_g_ESC_YawRate/1 -> ICAC/25(IMAPve_g_ESC_YawRate)
  IMAPve_d_ESC_YawRate_Valid/1 -> ICAC/26(IMAPve_d_ESC_YawRate_Valid)
  IMAPve_g_ESC_UnYawRate/1 -> ICAC/27(IMAPve_g_ESC_UnYawRate)
  IMAPve_g_ESC_VehSpd/1 -> ICAC/28(IMAPve_g_ESC_VehSpd)
  IMAPve_g_ESC_LonAcc/1 -> ICAC/29(IMAPve_g_ESC_LonAcc)
  IMAPve_d_ESC_LonAcc_Valid/1 -> ICAC/30(IMAPve_d_ESC_LonAcc_Valid)
  IMAPve_g_ESC_Brake_Press/1 -> ICAC/31(IMAPve_g_ESC_Brake_Press)
  IMAPve_g_ESC_Static_Slope/1 -> ICAC/32(IMAPve_g_ESC_Static_Slope)
  IMAPve_g_ESC_DySlope_Accuracy/1 -> ICAC/33(IMAPve_g_ESC_DySlope_Accuracy)
  IMAPve_g_ESC_DySlope/1 -> ICAC/34(IMAPve_g_ESC_DySlope)
  IMAPve_g_SW_Angle/1 -> ICAC/35(IMAPve_g_SW_Angle)
  IMAPve_g_SW_Angle_Speed/1 -> ICAC/36(IMAPve_g_SW_Angle_Speed)
  IMAPve_d_BCM_HazardLamp/1 -> ICAC/37(IMAPve_d_BCM_HazardLamp)
  IMAPve_d_BCM_Left_Light/1 -> ICAC/38(IMAPve_d_BCM_Left_Light)
  IMAPve_d_BCM_Right_Light/1 -> ICAC/39(IMAPve_d_BCM_Right_Light)
  IMAPve_d_ESC_BrakeLamp_Req/1 -> ICAC/40(IMAPve_d_ESC_BrakeLamp_Req)
  IMAPve_d_BCM_Opening_State/1 -> ICAC/41(IMAPve_d_BCM_Opening_State)
  IMAPve_d_BCM_Trunk_State/1 -> ICAC/42(IMAPve_d_BCM_Trunk_State)
  IMAPve_d_BCM_LF_Door_State/1 -> ICAC/43(IMAPve_d_BCM_LF_Door_State)
  IMAPve_d_BCM_RF_Door_State/1 -> ICAC/44(IMAPve_d_BCM_RF_Door_State)
  IMAPve_d_BCM_RR_Door_State/1 -> ICAC/45(IMAPve_d_BCM_RR_Door_State)
  IMAPve_d_BCM_LR_Door_State/1 -> ICAC/46(IMAPve_d_BCM_LR_Door_State)
  IMAPve_d_SCC_Left_SwitchSig/1 -> ICAC/47(IMAPve_d_SCC_Left_SwitchSig)
  IMAPve_d_SCC_Right_SwitchSig/1 -> ICAC/48(IMAPve_d_SCC_Right_SwitchSig)
  IMAPve_d_PEPS_Door_Lock_Req/1 -> ICAC/49(IMAPve_d_PEPS_Door_Lock_Req)
  IMAPve_d_BCM_Door_Lock_State/1 -> ICAC/50(IMAPve_d_BCM_Door_Lock_State)
  IMAPve_d_EMS_ACC_Status/1 -> ICAC/51(IMAPve_d_EMS_ACC_Status)
  IMAPve_g_EMS_Pot_WhlT_Max/1 -> ICAC/52(IMAPve_g_EMS_Pot_WhlT_Max)
  IMAPve_g_EMS_Pot_WhlT_Min/1 -> ICAC/53(IMAPve_g_EMS_Pot_WhlT_Min)
  IMAPve_g_EMS_RealPedal/1 -> ICAC/54(IMAPve_g_EMS_RealPedal)
  IMAPve_g_EMS_MaxTWhl/1 -> ICAC/55(IMAPve_g_EMS_MaxTWhl)
  IMAPve_g_EMS_MaxTWhl_Offset/1 -> ICAC/56(IMAPve_g_EMS_MaxTWhl_Offset)
  IMAPve_g_EMS_MinTWhl/1 -> ICAC/57(IMAPve_g_EMS_MinTWhl)
  IMAPve_g_EMS_MinTWhl_Offset/1 -> ICAC/58(IMAPve_g_EMS_MinTWhl_Offset)
  IMAPve_g_EMS_Actual_FlwT/1 -> ICAC/59(IMAPve_g_EMS_Actual_FlwT)
  IMAPve_g_EMS_Actual_IndT/1 -> ICAC/60(IMAPve_g_EMS_Actual_IndT)
  IMAPve_g_EMS_Realize_TWhl/1 -> ICAC/61(IMAPve_g_EMS_Realize_TWhl)
  IMAPve_g_EMS_ACC_VirtualPedal/1 -> ICAC/62(IMAPve_g_EMS_ACC_VirtualPedal)
  IMAPve_d_EMS_AccPedal_Fault/1 -> ICAC/63(IMAPve_d_EMS_AccPedal_Fault)
  IMAPve_g_EMS_Driver_Torque/1 -> ICAC/64(IMAPve_g_EMS_Driver_Torque)
  IMAPve_d_ESC_Brake_Effort/1 -> ICAC/65(IMAPve_d_ESC_Brake_Effort)
  IMAPve_g_EMS_Engine_Speed/1 -> ICAC/66(IMAPve_g_EMS_Engine_Speed)
  IMAPve_d_ESC_Veh_Standstill/1 -> ICAC/67(IMAPve_d_ESC_Veh_Standstill)
  IMAPve_d_TCU_Actual_Gear/1 -> ICAC/68(IMAPve_d_TCU_Actual_Gear)
  IMAPve_d_TCU_Target_Gear/1 -> ICAC/69(IMAPve_d_TCU_Target_Gear)
  IMAPve_d_TCU_PRND_State/1 -> ICAC/70(IMAPve_d_TCU_PRND_State)
  IMAPve_d_BCM_Ignition_State/1 -> ICAC/71(IMAPve_d_BCM_Ignition_State)
  IMAPve_d_ACU_Driver_Belt/1 -> ICAC/72(IMAPve_d_ACU_Driver_Belt)
  IMAPve_d_SWS_Fault_Code/1 -> ICAC/73(IMAPve_d_SWS_Fault_Code)
  IMAPve_d_SWS_Failure_Status/1 -> ICAC/74(IMAPve_d_SWS_Failure_Status)
  IMAPve_d_ESC_OFF/1 -> ICAC/75(IMAPve_d_ESC_OFF)
  IMAPve_d_ESC_AlarmSig/1 -> ICAC/76(IMAPve_d_ESC_AlarmSig)
  IMAPve_d_Speed_Limit_Switch/1 -> ICAC/77(IMAPve_d_Speed_Limit_Switch)
  IMAPve_d_ESC_ESC_Active/1 -> ICAC/78(IMAPve_d_ESC_ESC_Active)
  IMAPve_d_ESC_MSR_Active/1 -> ICAC/79(IMAPve_d_ESC_MSR_Active)
  IMAPve_d_ESC_TCS_Active/1 -> ICAC/80(IMAPve_d_ESC_TCS_Active)
  IMAPve_d_ESC_VehSpd_Valid/1 -> ICAC/81(IMAPve_d_ESC_VehSpd_Valid)
  IMAPve_d_Brake_Pedal_Fault/1 -> ICAC/82(IMAPve_d_Brake_Pedal_Fault)
  IMAPve_d_ESC_ABS_Active/1 -> ICAC/83(IMAPve_d_ESC_ABS_Active)
  IMAPve_d_ESC_ABS_Valid/1 -> ICAC/84(IMAPve_d_ESC_ABS_Valid)
  IMAPve_d_ESC_ABS_AlarmSig/1 -> ICAC/85(IMAPve_d_ESC_ABS_AlarmSig)
  IMAPve_d_ESC_FL_WheelPulVal/1 -> ICAC/86(IMAPve_d_ESC_FL_WheelPulVal)
  IMAPve_d_ESC_FR_WheelPulVal/1 -> ICAC/87(IMAPve_d_ESC_FR_WheelPulVal)
  IMAPve_d_ESC_RL_WheelPulVal/1 -> ICAC/88(IMAPve_d_ESC_RL_WheelPulVal)
  IMAPve_d_ESC_RR_WheelPulVal/1 -> ICAC/89(IMAPve_d_ESC_RR_WheelPulVal)
  IMAPve_g_ESC_FL_WhlSpd/1 -> ICAC/90(IMAPve_g_ESC_FL_WhlSpd)
  IMAPve_d_ESC_FL_WhlSpd_Fault/1 -> ICAC/91(IMAPve_d_ESC_FL_WhlSpd_Fault)
  IMAPve_g_ESC_FR_WhlSpd/1 -> ICAC/92(IMAPve_g_ESC_FR_WhlSpd)
  IMAPve_d_ESC_FR_WhlSpd_Fault/1 -> ICAC/93(IMAPve_d_ESC_FR_WhlSpd_Fault)
  IMAPve_g_ESC_RL_WhlSpd/1 -> ICAC/94(IMAPve_g_ESC_RL_WhlSpd)
  IMAPve_d_ESC_RL_WhlSpd_Fault/1 -> ICAC/95(IMAPve_d_ESC_RL_WhlSpd_Fault)
  IMAPve_g_ESC_RR_WhlSpd/1 -> ICAC/96(IMAPve_g_ESC_RR_WhlSpd)
  IMAPve_d_ESC_RR_WhlSpd_Fault/1 -> ICAC/97(IMAPve_d_ESC_RR_WhlSpd_Fault)
  IMAPve_d_ESC_FL_Wheel_Pulse/1 -> ICAC/98(IMAPve_d_ESC_FL_Wheel_Pulse)
  IMAPve_d_ESC_FR_Wheel_Pulse/1 -> ICAC/99(IMAPve_d_ESC_FR_Wheel_Pulse)
  IMAPve_d_ESC_RL_Wheel_Pulse/1 -> ICAC/100(IMAPve_d_ESC_RL_Wheel_Pulse)
  IMAPve_d_ESC_RR_Wheel_Pulse/1 -> ICAC/101(IMAPve_d_ESC_RR_Wheel_Pulse)
  IMAPve_d_TCU_AT_Failure/1 -> ICAC/102(IMAPve_d_TCU_AT_Failure)
  IMAPve_d_TCU_Shift_Valid/1 -> ICAC/103(IMAPve_d_TCU_Shift_Valid)
  IMAPve_d_TCU_DCT_Clutch_State/1 -> ICAC/104(IMAPve_d_TCU_DCT_Clutch_State)
  IMAPve_d_TCU_Gear_Engage/1 -> ICAC/105(IMAPve_d_TCU_Gear_Engage)
  IMAPve_d_TCU_Select_ATMode/1 -> ICAC/106(IMAPve_d_TCU_Select_ATMode)
  IMAPve_d_EMS_Engine_Status/1 -> ICAC/107(IMAPve_d_EMS_Engine_Status)
  IMAPve_d_EMS_Gearbox_CtlAvail/1 -> ICAC/108(IMAPve_d_EMS_Gearbox_CtlAvail)
  IMAPve_d_ESC_Brake_Failsafe/1 -> ICAC/109(IMAPve_d_ESC_Brake_Failsafe)
  IMAPve_d_ESC_AEB_Status/1 -> ICAC/110(IMAPve_d_ESC_AEB_Status)
  IMAPve_d_ESC_AEB_Available/1 -> ICAC/111(IMAPve_d_ESC_AEB_Available)
  IMAPve_d_ESC_AEB_Active/1 -> ICAC/112(IMAPve_d_ESC_AEB_Active)
  IMAPve_d_ESC_ACC_Status/1 -> ICAC/113(IMAPve_d_ESC_ACC_Status)
  IMAPve_d_ESC_ACC_Available/1 -> ICAC/114(IMAPve_d_ESC_ACC_Available)
  IMAPve_d_ESC_ACC_Active/1 -> ICAC/115(IMAPve_d_ESC_ACC_Active)
  IMAPve_d_EMS_ACC_Effective/1 -> ICAC/116(IMAPve_d_EMS_ACC_Effective)
  IMAPve_d_BCM_FrontWiper_State/1 -> ICAC/117(IMAPve_d_BCM_FrontWiper_State)
  IMAPve_d_BCM_CHMSL_Status/1 -> ICAC/118(IMAPve_d_BCM_CHMSL_Status)
  IMAPve_d_BCM_BrakeLamp_State/1 -> ICAC/119(IMAPve_d_BCM_BrakeLamp_State)
  IMAPve_d_GW_Brake_Only_Req/1 -> ICAC/120(IMAPve_d_GW_Brake_Only_Req)
  IMAPve_d_ACU_Passenger_Belt/1 -> ICAC/121(IMAPve_d_ACU_Passenger_Belt)
  IMAPve_d_EMS_ACC_CtlAvail/1 -> ICAC/122(IMAPve_d_EMS_ACC_CtlAvail)
  IMAPve_d_EMS_ACC_Inhibited/1 -> ICAC/123(IMAPve_d_EMS_ACC_Inhibited)
  IMAPve_d_EMS_Brake_Pedal/1 -> ICAC/124(IMAPve_d_EMS_Brake_Pedal)
  IMAPve_d_BCM_LowBeam_State/1 -> ICAC/125(IMAPve_d_BCM_LowBeam_State)
  IMAPve_d_BCM_HighBeam_State/1 -> ICAC/126(IMAPve_d_BCM_HighBeam_State)
  IMAPve_d_EPB_Status/1 -> ICAC/127(IMAPve_d_EPB_Status)
  IMAPve_d_EPB_Display_Req/1 -> ICAC/128(IMAPve_d_EPB_Display_Req)
  IMAPve_d_EPB_Warn_Req/1 -> ICAC/129(IMAPve_d_EPB_Warn_Req)
  IMAPve_d_EPB_Switch_State/1 -> ICAC/130(IMAPve_d_EPB_Switch_State)
  IMAPve_d_EPB_Switch_Valid/1 -> ICAC/131(IMAPve_d_EPB_Switch_Valid)
  IMAPve_d_ESC_Drive_Direction/1 -> ICAC/132(IMAPve_d_ESC_Drive_Direction)
  IMAPve_d_ESC_Hold_State/1 -> ICAC/133(IMAPve_d_ESC_Hold_State)
  IMAPve_d_EPS_Steer_Hold_State/1 -> ICAC/134(IMAPve_d_EPS_Steer_Hold_State)
  IMAPve_d_EPS_Warning_State/1 -> ICAC/135(IMAPve_d_EPS_Warning_State)
  IMAPve_g_EPS_PowerCon/1 -> ICAC/136(IMAPve_g_EPS_PowerCon)
  IMAPve_d_ESC_EBD_AlarmSig/1 -> ICAC/137(IMAPve_d_ESC_EBD_AlarmSig)
  IMAPve_d_ESC_AVH_Status/1 -> ICAC/138(IMAPve_d_ESC_AVH_Status)
  IMAPve_d_Radar_Detective_Req/1 -> ICAC/139(IMAPve_d_Radar_Detective_Req)
  IMAPve_g_BCM_Battery_Voltage/1 -> ICAC/140(IMAPve_g_BCM_Battery_Voltage)
  IMAPve_d_TBOX_LocalTimeY/1 -> ICAC/141(IMAPve_d_TBOX_LocalTimeY)
  IMAPve_d_TBOX_LocalTimeM/1 -> ICAC/142(IMAPve_d_TBOX_LocalTimeM)
  IMAPve_d_TBOX_LocalTimeD/1 -> ICAC/143(IMAPve_d_TBOX_LocalTimeD)
  IMAPve_d_TBOX_LocalTimeH/1 -> ICAC/144(IMAPve_d_TBOX_LocalTimeH)
  IMAPve_d_TBOX_LocalTimeMin/1 -> ICAC/145(IMAPve_d_TBOX_LocalTimeMin)
  IMAPve_d_TBOX_LocalTimeS/1 -> ICAC/146(IMAPve_d_TBOX_LocalTimeS)
  IMAPve_d_TBOX_LocalTime_Valid/1 -> ICAC/147(IMAPve_d_TBOX_LocalTime_Valid)
  IMAPve_d_TPMS_Warn_Indicate/1 -> ICAC/148(IMAPve_d_TPMS_Warn_Indicate)
  IMAPve_d_Radar_State/1 -> ICAC/149(IMAPve_d_Radar_State)
  IMAPve_d_ACC_Desired_Headway/1 -> ICAC/150(IMAPve_d_ACC_Desired_Headway)
  IMAPve_d_Time_System_Clock/1 -> ICAC/151(IMAPve_d_Time_System_Clock)
  IMAPve_d_Signal_Time_Stamp/1 -> ICAC/152(IMAPve_d_Signal_Time_Stamp)
  IMAPve_g_GW_IC_Odometer/1 -> ICAC/153(IMAPve_g_GW_IC_Odometer)
  IMAPve_g_FAPA_State/1 -> ICAC/154(IMAPve_g_FAPA_State)
  IMAPve_d_Outside_Temp/1 -> ICAC/155(IMAPve_d_Outside_Temp)
  IMAPve_d_ORI_CIPV_ID/1 -> ICAC/156(IMAPve_d_ORI_CIPV_ID)
  IMAPve_d_ORI_Obj_Num/1 -> ICAC/157(IMAPve_d_ORI_Obj_Num)
  IMAPva_g_ORI_Probability/1 -> ICAC/158(IMAPva_g_ORI_Probability)
  IMAPva_d_ORI_Obj_Class/1 -> ICAC/159(IMAPva_d_ORI_Obj_Class)
  IMAPva_d_ORI_Obj_Motion/1 -> ICAC/160(IMAPva_d_ORI_Obj_Motion)
  IMAPva_g_ORI_Obj_RelVel/1 -> ICAC/161(IMAPva_g_ORI_Obj_RelVel)
  IMAPva_g_ORI_Obj_LongDis/1 -> ICAC/162(IMAPva_g_ORI_Obj_LongDis)
  IMAPva_d_ORI_Obj_Lane/1 -> ICAC/163(IMAPva_d_ORI_Obj_Lane)
  IMAPva_g_ORI_Obj_LAngle/1 -> ICAC/164(IMAPva_g_ORI_Obj_LAngle)
  IMAPva_g_ORI_Obj_RAngle/1 -> ICAC/165(IMAPva_g_ORI_Obj_RAngle)
  IMAPva_g_ORI_Obj_Width/1 -> ICAC/166(IMAPva_g_ORI_Obj_Width)
  IMAPva_d_ORI_Obj_ID/1 -> ICAC/167(IMAPva_d_ORI_Obj_ID)
  IMAPve_d_ORI_Lane_Valid/1 -> ICAC/168(IMAPve_d_ORI_Lane_Valid)
  IMAPve_d_ORI_Lane_ConsArea/1 -> ICAC/169(IMAPve_d_ORI_Lane_ConsArea)
  IMAPve_d_ORI_Lane_RoadType/1 -> ICAC/170(IMAPve_d_ORI_Lane_RoadType)
  IMAPve_g_ORI_L0_C3/1 -> ICAC/171(IMAPve_g_ORI_L0_C3)
  IMAPve_g_ORI_L0_C2/1 -> ICAC/172(IMAPve_g_ORI_L0_C2)
  IMAPve_g_ORI_L0_C1/1 -> ICAC/173(IMAPve_g_ORI_L0_C1)
  IMAPve_g_ORI_L0_C0/1 -> ICAC/174(IMAPve_g_ORI_L0_C0)
  IMAPve_d_ORI_L0_Q/1 -> ICAC/175(IMAPve_d_ORI_L0_Q)
  IMAPve_d_ORI_L0_Type/1 -> ICAC/176(IMAPve_d_ORI_L0_Type)
  IMAPve_g_ORI_L0_VR/1 -> ICAC/177(IMAPve_g_ORI_L0_VR)
  IMAPve_g_ORI_L0_TLC/1 -> ICAC/178(IMAPve_g_ORI_L0_TLC)
  IMAPve_g_ORI_L0_W/1 -> ICAC/179(IMAPve_g_ORI_L0_W)
  IMAPve_d_ORI_L0_LC/1 -> ICAC/180(IMAPve_d_ORI_L0_LC)
  IMAPve_g_ORI_L1_C3/1 -> ICAC/181(IMAPve_g_ORI_L1_C3)
  IMAPve_g_ORI_L1_C2/1 -> ICAC/182(IMAPve_g_ORI_L1_C2)
  IMAPve_g_ORI_L1_C1/1 -> ICAC/183(IMAPve_g_ORI_L1_C1)
  IMAPve_g_ORI_L1_C0/1 -> ICAC/184(IMAPve_g_ORI_L1_C0)
  IMAPve_d_ORI_L1_Q/1 -> ICAC/185(IMAPve_d_ORI_L1_Q)
  IMAPve_d_ORI_L1_Type/1 -> ICAC/186(IMAPve_d_ORI_L1_Type)
  IMAPve_g_ORI_L1_VR/1 -> ICAC/187(IMAPve_g_ORI_L1_VR)
  IMAPve_g_ORI_L1_TLC/1 -> ICAC/188(IMAPve_g_ORI_L1_TLC)
  IMAPve_g_ORI_L1_W/1 -> ICAC/189(IMAPve_g_ORI_L1_W)
  IMAPve_d_ORI_L1_LC/1 -> ICAC/190(IMAPve_d_ORI_L1_LC)
  IMAPve_g_ORI_R0_C3/1 -> ICAC/191(IMAPve_g_ORI_R0_C3)
  IMAPve_g_ORI_R0_C2/1 -> ICAC/192(IMAPve_g_ORI_R0_C2)
  IMAPve_g_ORI_R0_C1/1 -> ICAC/193(IMAPve_g_ORI_R0_C1)
  IMAPve_g_ORI_R0_C0/1 -> ICAC/194(IMAPve_g_ORI_R0_C0)
  IMAPve_d_ORI_R0_Q/1 -> ICAC/195(IMAPve_d_ORI_R0_Q)
  IMAPve_d_ORI_R0_LT/1 -> ICAC/196(IMAPve_d_ORI_R0_LT)
  IMAPve_g_ORI_R0_VR/1 -> ICAC/197(IMAPve_g_ORI_R0_VR)
  IMAPve_g_ORI_R0_TLC/1 -> ICAC/198(IMAPve_g_ORI_R0_TLC)
  IMAPve_g_ORI_R0_W/1 -> ICAC/199(IMAPve_g_ORI_R0_W)
  IMAPve_d_ORI_R0_LC/1 -> ICAC/200(IMAPve_d_ORI_R0_LC)
  IMAPve_g_ORI_R1_C3/1 -> ICAC/201(IMAPve_g_ORI_R1_C3)
  IMAPve_g_ORI_R1_C2/1 -> ICAC/202(IMAPve_g_ORI_R1_C2)
  IMAPve_g_ORI_R1_C1/1 -> ICAC/203(IMAPve_g_ORI_R1_C1)
  IMAPve_g_ORI_R1_C0/1 -> ICAC/204(IMAPve_g_ORI_R1_C0)
  IMAPve_d_ORI_R1_Q/1 -> ICAC/205(IMAPve_d_ORI_R1_Q)
  IMAPve_d_ORI_R1_LT/1 -> ICAC/206(IMAPve_d_ORI_R1_LT)
  IMAPve_g_ORI_R1_VR/1 -> ICAC/207(IMAPve_g_ORI_R1_VR)
  IMAPve_g_ORI_R1_TLC/1 -> ICAC/208(IMAPve_g_ORI_R1_TLC)
  IMAPve_g_ORI_R1_W/1 -> ICAC/209(IMAPve_g_ORI_R1_W)
  IMAPve_d_ORI_R1_LC/1 -> ICAC/210(IMAPve_d_ORI_R1_LC)
  IMAPve_d_Sensor_Status/1 -> ICAC/211(IMAPve_d_Sensor_Status)
  IMAPve_d_LF_Radar_Status/1 -> ICAC/212(IMAPve_d_LF_Radar_Status)
  IMAPve_d_RF_Radar_Status/1 -> ICAC/213(IMAPve_d_RF_Radar_Status)
  IMAPve_d_LR_Radar_Status/1 -> ICAC/214(IMAPve_d_LR_Radar_Status)
  IMAPve_d_RR_Radar_Status/1 -> ICAC/215(IMAPve_d_RR_Radar_Status)
  IMAPve_d_Fusion_Status/1 -> ICAC/216(IMAPve_d_Fusion_Status)
  IMAPve_g_Fusion_Time_Stamp/1 -> ICAC/217(IMAPve_g_Fusion_Time_Stamp)
  IMAPve_d_obj_Num/1 -> ICAC/218(IMAPve_d_obj_Num)
  IMAPva_d_obj_id/1 -> ICAC/219(IMAPva_d_obj_id)
  IMAPva_g_obj_pos_x/1 -> ICAC/220(IMAPva_g_obj_pos_x)
  IMAPva_g_obj_pos_y/1 -> ICAC/221(IMAPva_g_obj_pos_y)
  IMAPva_g_obj_vel_x/1 -> ICAC/222(IMAPva_g_obj_vel_x)
  IMAPva_g_obj_vel_y/1 -> ICAC/223(IMAPva_g_obj_vel_y)
  IMAPva_g_obj_acc_x/1 -> ICAC/224(IMAPva_g_obj_acc_x)
  IMAPva_g_obj_acc_y/1 -> ICAC/225(IMAPva_g_obj_acc_y)
  IMAPva_g_obj_pos_var_x/1 -> ICAC/226(IMAPva_g_obj_pos_var_x)
  IMAPva_g_obj_pos_var_y/1 -> ICAC/227(IMAPva_g_obj_pos_var_y)
  IMAPva_g_obj_pos_var_xy/1 -> ICAC/228(IMAPva_g_obj_pos_var_xy)
  IMAPva_g_obj_vel_var_x/1 -> ICAC/229(IMAPva_g_obj_vel_var_x)
  IMAPva_g_obj_vel_var_y/1 -> ICAC/230(IMAPva_g_obj_vel_var_y)
  IMAPva_g_obj_vel_var_xy/1 -> ICAC/231(IMAPva_g_obj_vel_var_xy)
  IMAPva_g_obj_width/1 -> ICAC/232(IMAPva_g_obj_width)
  IMAPva_g_obj_length/1 -> ICAC/233(IMAPva_g_obj_length)
  IMAPva_d_obj_fusion_type/1 -> ICAC/234(IMAPva_d_obj_fusion_type)
  IMAPva_d_obj_class/1 -> ICAC/235(IMAPva_d_obj_class)
  IMAPva_d_obj_lane/1 -> ICAC/236(IMAPva_d_obj_lane)
  IMAPva_d_obj_status/1 -> ICAC/237(IMAPva_d_obj_status)
  IMAPva_d_obj_cam_asso_id/1 -> ICAC/238(IMAPva_d_obj_cam_asso_id)
  IMAPva_g_obj_con/1 -> ICAC/239(IMAPva_g_obj_con)
  IMAPva_g_obj_age/1 -> ICAC/240(IMAPva_g_obj_age)
  IMAPva_d_obj_TurnLight/1 -> ICAC/241(IMAPva_d_obj_TurnLight)
  IMAPva_d_obj_BrakeLight/1 -> ICAC/242(IMAPva_d_obj_BrakeLight)
  IMAPva_d_obj_MotionStatus/1 -> ICAC/243(IMAPva_d_obj_MotionStatus)
  IMAPva_d_obj_ACC/1 -> ICAC/244(IMAPva_d_obj_ACC)
  IMAPva_d_obj_AEB/1 -> ICAC/245(IMAPva_d_obj_AEB)
  IMAPva_d_obj_ELK/1 -> ICAC/246(IMAPva_d_obj_ELK)
  IMAPva_d_obj_ALC/1 -> ICAC/247(IMAPva_d_obj_ALC)
  IMAPva_d_obj_ESA/1 -> ICAC/248(IMAPva_d_obj_ESA)
  IMAPva_d_obj_JA/1 -> ICAC/249(IMAPva_d_obj_JA)
  IMAPve_d_Lane_Valid/1 -> ICAC/250(IMAPve_d_Lane_Valid)
  IMAPve_d_Road_Type/1 -> ICAC/251(IMAPve_d_Road_Type)
  IMAPve_d_ConsArea/1 -> ICAC/252(IMAPve_d_ConsArea)
  IMAPve_g_L0_C0/1 -> ICAC/253(IMAPve_g_L0_C0)
  IMAPve_g_L0_C1/1 -> ICAC/254(IMAPve_g_L0_C1)
  IMAPve_g_L0_C2/1 -> ICAC/255(IMAPve_g_L0_C2)
  IMAPve_g_L0_C3/1 -> ICAC/256(IMAPve_g_L0_C3)
  IMAPve_g_L0_VR/1 -> ICAC/257(IMAPve_g_L0_VR)
  IMAPve_d_L0_Q/1 -> ICAC/258(IMAPve_d_L0_Q)
  IMAPve_d_L0_Type/1 -> ICAC/259(IMAPve_d_L0_Type)
  IMAPve_g_L0_Confidence/1 -> ICAC/260(IMAPve_g_L0_Confidence)
  IMAPve_g_L0_W/1 -> ICAC/261(IMAPve_g_L0_W)
  IMAPve_g_L0_TLC/1 -> ICAC/262(IMAPve_g_L0_TLC)
  IMAPve_d_L0_LC/1 -> ICAC/263(IMAPve_d_L0_LC)
  IMAPve_g_R0_C0/1 -> ICAC/264(IMAPve_g_R0_C0)
  IMAPve_g_R0_C1/1 -> ICAC/265(IMAPve_g_R0_C1)
  IMAPve_g_R0_C2/1 -> ICAC/266(IMAPve_g_R0_C2)
  IMAPve_g_R0_C3/1 -> ICAC/267(IMAPve_g_R0_C3)
  IMAPve_g_R0_VR/1 -> ICAC/268(IMAPve_g_R0_VR)
  IMAPve_d_R0_Q/1 -> ICAC/269(IMAPve_d_R0_Q)
  IMAPve_d_R0_Type/1 -> ICAC/270(IMAPve_d_R0_Type)
  IMAPve_g_R0_Confidence/1 -> ICAC/271(IMAPve_g_R0_Confidence)
  IMAPve_g_R0_W/1 -> ICAC/272(IMAPve_g_R0_W)
  IMAPve_g_R0_TLC/1 -> ICAC/273(IMAPve_g_R0_TLC)
  IMAPve_d_R0_LC/1 -> ICAC/274(IMAPve_d_R0_LC)
  IMAPve_g_L1_C0/1 -> ICAC/275(IMAPve_g_L1_C0)
  IMAPve_g_L1_C1/1 -> ICAC/276(IMAPve_g_L1_C1)
  IMAPve_g_L1_C2/1 -> ICAC/277(IMAPve_g_L1_C2)
  IMAPve_g_L1_C3/1 -> ICAC/278(IMAPve_g_L1_C3)
  IMAPve_g_L1_VR/1 -> ICAC/279(IMAPve_g_L1_VR)
  IMAPve_d_L1_Q/1 -> ICAC/280(IMAPve_d_L1_Q)
  IMAPve_d_L1_Type/1 -> ICAC/281(IMAPve_d_L1_Type)
  IMAPve_g_L1_Confidence/1 -> ICAC/282(IMAPve_g_L1_Confidence)
  IMAPve_g_L1_W/1 -> ICAC/283(IMAPve_g_L1_W)
  IMAPve_g_L1_TLC/1 -> ICAC/284(IMAPve_g_L1_TLC)
  IMAPve_d_L1_LC/1 -> ICAC/285(IMAPve_d_L1_LC)
  IMAPve_g_R1_C0/1 -> ICAC/286(IMAPve_g_R1_C0)
  IMAPve_g_R1_C1/1 -> ICAC/287(IMAPve_g_R1_C1)
  IMAPve_g_R1_C2/1 -> ICAC/288(IMAPve_g_R1_C2)
  IMAPve_g_R1_C3/1 -> ICAC/289(IMAPve_g_R1_C3)
  IMAPve_g_R1_VR/1 -> ICAC/290(IMAPve_g_R1_VR)
  IMAPve_d_R1_Q/1 -> ICAC/291(IMAPve_d_R1_Q)
  IMAPve_d_R1_Type/1 -> ICAC/292(IMAPve_d_R1_Type)
  IMAPve_g_R1_Confidence/1 -> ICAC/293(IMAPve_g_R1_Confidence)
  IMAPve_g_R1_W/1 -> ICAC/294(IMAPve_g_R1_W)
  IMAPve_g_R1_TLC/1 -> ICAC/295(IMAPve_g_R1_TLC)
  IMAPve_d_R1_LC/1 -> ICAC/296(IMAPve_d_R1_LC)
  IMAPve_g_L0_C0_Back/1 -> ICAC/297(IMAPve_g_L0_C0_Back)
  IMAPve_g_L0_C1_Back/1 -> ICAC/298(IMAPve_g_L0_C1_Back)
  IMAPve_g_L0_C2_Back/1 -> ICAC/299(IMAPve_g_L0_C2_Back)
  IMAPve_g_L0_C3_Back/1 -> ICAC/300(IMAPve_g_L0_C3_Back)
  IMAPve_g_L0_Range_Back/1 -> ICAC/301(IMAPve_g_L0_Range_Back)
  IMAPve_g_L0_C0_FR_Pred/1 -> ICAC/302(IMAPve_g_L0_C0_FR_Pred)
  IMAPve_g_L0_C1_FR_Pred/1 -> ICAC/303(IMAPve_g_L0_C1_FR_Pred)
  IMAPve_g_L0_C2_FR_Pred/1 -> ICAC/304(IMAPve_g_L0_C2_FR_Pred)
  IMAPve_g_L0_Range_FR_Pred/1 -> ICAC/305(IMAPve_g_L0_Range_FR_Pred)
  IMAPve_g_R0_C0_Back/1 -> ICAC/306(IMAPve_g_R0_C0_Back)
  IMAPve_g_R0_C1_Back/1 -> ICAC/307(IMAPve_g_R0_C1_Back)
  IMAPve_g_R0_C2_Back/1 -> ICAC/308(IMAPve_g_R0_C2_Back)
  IMAPve_g_R0_C3_Back/1 -> ICAC/309(IMAPve_g_R0_C3_Back)
  IMAPve_g_R0_Range_Back/1 -> ICAC/310(IMAPve_g_R0_Range_Back)
  IMAPve_g_R0_C0_FR_Pred/1 -> ICAC/311(IMAPve_g_R0_C0_FR_Pred)
  IMAPve_g_R0_C1_FR_Pred/1 -> ICAC/312(IMAPve_g_R0_C1_FR_Pred)
  IMAPve_g_R0_C2_FR_Pred/1 -> ICAC/313(IMAPve_g_R0_C2_FR_Pred)
  IMAPve_g_R0_Range_FR_Pred/1 -> ICAC/314(IMAPve_g_R0_Range_FR_Pred)
  IMAPve_g_L1_C0_Back/1 -> ICAC/315(IMAPve_g_L1_C0_Back)
  IMAPve_g_L1_C1_Back/1 -> ICAC/316(IMAPve_g_L1_C1_Back)
  IMAPve_g_L1_C2_Back/1 -> ICAC/317(IMAPve_g_L1_C2_Back)
  IMAPve_g_L1_C3_Back/1 -> ICAC/318(IMAPve_g_L1_C3_Back)
  IMAPve_g_L1_Range_Back/1 -> ICAC/319(IMAPve_g_L1_Range_Back)
  IMAPve_g_L1_C0_FR_Pred/1 -> ICAC/320(IMAPve_g_L1_C0_FR_Pred)
  IMAPve_g_L1_C1_FR_Pred/1 -> ICAC/321(IMAPve_g_L1_C1_FR_Pred)
  IMAPve_g_L1_C2_FR_Pred/1 -> ICAC/322(IMAPve_g_L1_C2_FR_Pred)
  IMAPve_g_L1_Range_FR_Pred/1 -> ICAC/323(IMAPve_g_L1_Range_FR_Pred)
  IMAPve_g_R1_C0_Back/1 -> ICAC/324(IMAPve_g_R1_C0_Back)
  IMAPve_g_R1_C1_Back/1 -> ICAC/325(IMAPve_g_R1_C1_Back)
  IMAPve_g_R1_C2_Back/1 -> ICAC/326(IMAPve_g_R1_C2_Back)
  IMAPve_g_R1_C3_Back/1 -> ICAC/327(IMAPve_g_R1_C3_Back)
  IMAPve_g_R1_Range_Back/1 -> ICAC/328(IMAPve_g_R1_Range_Back)
  IMAPve_g_R1_C0_FR_Pred/1 -> ICAC/329(IMAPve_g_R1_C0_FR_Pred)
  IMAPve_g_R1_C1_FR_Pred/1 -> ICAC/330(IMAPve_g_R1_C1_FR_Pred)
  IMAPve_g_R1_C2_FR_Pred/1 -> ICAC/331(IMAPve_g_R1_C2_FR_Pred)
  IMAPve_g_R1_Range_FR_Pred/1 -> ICAC/332(IMAPve_g_R1_Range_FR_Pred)
  IMAPve_d_Sign_ISA_Value/1 -> ICAC/333(IMAPve_d_Sign_ISA_Value)
  IMAPve_d_TSR_Sign_Type/1 -> ICAC/334(IMAPve_d_TSR_Sign_Type)
  IMAPve_d_Camera_Signal_Fault/1 -> ICAC/335(IMAPve_d_Camera_Signal_Fault)
  IMAPve_d_Radar_Status/1 -> ICAC/336(IMAPve_d_Radar_Status)
  IMAPve_d_Camera_Status/1 -> ICAC/337(IMAPve_d_Camera_Status)
  Runnable_ICAC_Step/1 -> ICAC/Trigger
  ICAC/1(ICACve_g_SteerAngleCmd) -> ICACve_g_SteerAngleCmd/1
  ICAC/2(ICACve_d_SteerAngleVld) -> ICACve_d_SteerAngleVld/1
  ICAC/3(ICACve_d_SignalTStamp) -> ICACve_d_SignalTStamp/1
